simulink model "AUV_Multi_MPC"  (R2023a)
settings: Solver=ode23t  StartTime=0.0  StopTime=300  MaxStep=0.01  RelTol=1e-3  EnableMultiTasking=on
PreLoadFcn:
  | AUV_VehicleParameters;
  | Vehicle.Body.markeropacity = 0;
InitFcn:
  | %% ========================= SAMPLE TIME =========================
  | Ts = 0.1;
  | %% ========================= MPC: SURGE X =========================
  | nx = 1; nu = 1; ny = 1;
  | 
  | A = 0.9; B = 0.1; C = 1; D = 0;
  | plant = ss(A, B, C, D, Ts);
  | mpc1 = mpc(plant, Ts);
  | 
  | % Cấu hình như bình thường
  | mpc1.PredictionHorizon = 10;
  | mpc1.ControlHorizon = 2;
  | 
  | mpc1.Weights.OV = 7.5; % đủ mạnh để bám
  | mpc1.Weights.MV = 0.08; % cho dùng lực nhiều hơn
  | mpc1.Weights.MVRate = 0.25; % vừa mượt vừa linh hoạt
  | mpc1.MV.Min = -40;
  | mpc1.MV.Max = 40;
  | mpc1.OV.Min = 0;
  | mpc1.OV.Max = 2;
  | 
  | % Ràng buộc về thay đổi lực
  | mpc1.MV.RateMin = -12.5;
  | mpc1.MV.RateMax = 12.5;
  | %% ========================= MPC OUTER LOOP FOR DEPTH (Z) =========================
  | % ===== Baseline outer MPC for depth =====
  | u0 = 1.2;
  | 
  | A = 1;
  | B = -Ts*u0;
  | C = 1;
  | D = 0;
  | 
  | plant_z = ss(A,B,C,D,Ts);
  | 
  | mpc_z = mpc(plant_z,Ts);
  | mpc_z.PredictionHorizon = 10;
  | mpc_z.ControlHorizon    = 2;
  | 
  | mpc_z.Weights.OV     = 12;
  | mpc_z.Weights.MV     = 0.01;
  | mpc_z.Weights.MVRate = 0.1;
  | 
  | theta_ref_max = deg2rad(18);
  | mpc_z.MV.Min = -theta_ref_max;
  | mpc_z.MV.Max =  theta_ref_max;
  | 
  | mpc_z.MV.RateMin = -deg2rad(4);
  | mpc_z.MV.RateMax =  deg2rad(4);
  | 
  | 
  | %% ========================= MPC OUTER LOOP FOR HEADING =========================
  | A = 1;
  | B = Ts;
  | C = 1;
  | D = 0;
  | 
  | plant_psi = ss(A,B,C,D,Ts);
  | mpc_psi = mpc(plant_psi,Ts);
  | 
  | ... (+13 lines)
StopFcn:
  | try
  |     S = out;
  | 
  |     % ===============================
  |     % CHỌN HỆ QUY CHIẾU
  |     % ===============================
  |     USE_UP = true;   % true = ENU (Up), false = NED (Down)
  | 
  |     % ===============================
  |     % AUV position (NED gốc)
  |     % ===============================
  |     P  = squeeze(S.auv_position.signals.values);   % [Xn Ye Zd]
  |     tP = S.auv_position.time(:);
  | 
  |     Xn = P(:,1);   % North
  |     Ye = P(:,2);   % East
  |     Zd = P(:,3);   % Down (+)
  | 
  |     % ===============================
  |     % Reference vector
  |     % ===============================
  |     R = squeeze(S.auv_reference.signals.values);  % [V D psi]
  |     t = S.auv_reference.time(:);
  | 
  |     V   = R(:,1);      % speed
  |     D   = R(:,2);      % depth (Down +)
  |     psi = R(:,3);      % heading (rad)
  | 
  |     % ===============================
  |     % Reconstruct reference trajectory (NED)
  |     % ===============================
  |     Xr = Xn(1) + cumtrapz(t, V .* cos(psi));   % North
  |     Yr = Ye(1) + cumtrapz(t, V .* sin(psi));   % East
  |     Zr_down = Zd(1) + (D - D(1));              % Down (+)
  | 
  |     % ===============================
  |     % CHUYỂN HỆ (nếu cần)
  |     % ===============================
  |     if USE_UP
  |         Za  = -Zd;        % Up
  |         Zr  = -Zr_down;   % Up
  |         zlbl = 'Z (Up, m)';
  |     else
  |         Za  = Zd;         % Down
  |         Zr  = Zr_down;
  |         zlbl = 'Z (Down, m)';
  |     end
  | 
  |     % ===============================
  |     % Plot
  |     % ===============================
  |     f = figure(2); clf(f);
  |     set(f,'Name','AUV vs Reference','NumberTitle','off');
  | 
  |     ax = gca;
  |     ax.SortMethod = 'childorder';
  | 
  |     hRef   = plot3(Xr, Yr, Zr, '--', ...
  |                    'Color',[0.6 0.6 0.6], 'LineWidth',1.2);
  |     hold on
  | ... (+24 lines)
model workspace: external: MATLAB File AUV_DataFile_ORIG.m (data not in the file)
undefined symbols (not defined in the file): Environment, Multibody, Newton, Raphson, smiData, X, x, Y, y, Z
libraries: sm_lib x3123, nesl_utility x51, sharedutil x8, simulink x6, AUVCustomPrimitives_Lib x4, mpclib x3, fuzblock x2, instrumentseriallib x2, shared6dof x1, slpidlib x1, aerolibasang x1, aerolibadyn x1
(part 7 of 72)

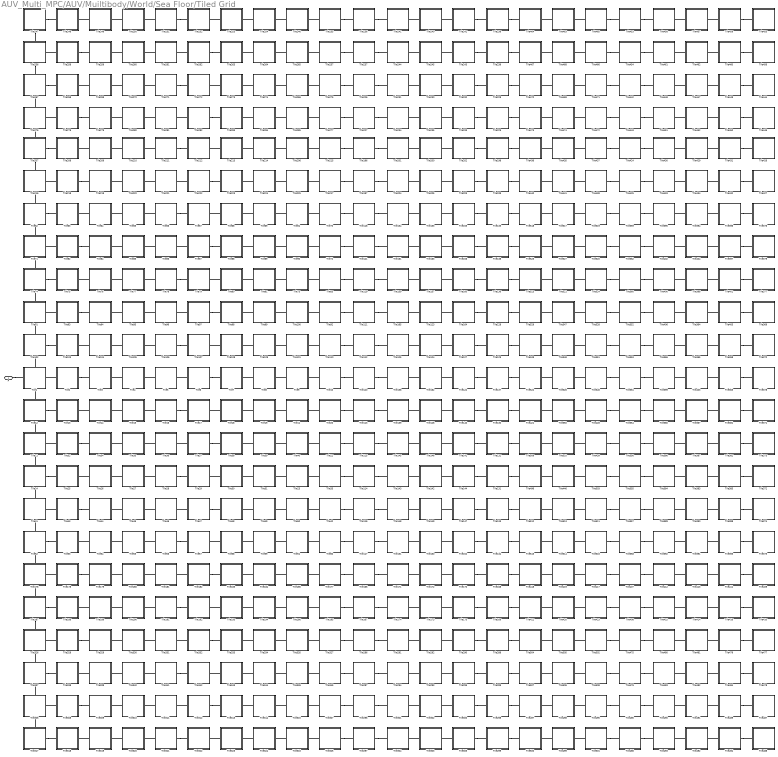
== system AUV_Multi_MPC/AUV/Muiltibody/World/Sea Floor/Tiled Grid ==
  Tile1 : Subsystem  mask(Square Tile){side=side, thickness=thick, color=color1, opacity=opacity}
      mask prompts: side "Side (m) :"; thickness "Thickness (m) :"; color "Color [RGB] :"; opacity "Opacity (0...1) :"
      mask help: This block creates a flat, single, square tile element. The square tile body is mass-less, so it will not have an effect on the dynamic simulation. This square tile element can be used as a graphic reference by itself, or as part of a composite graphic reference made of an array of interconnected tiles. The square tile is aligned with the XY plane, and the block provides frame connector ports to the middle points on each of the four sides of the body of the square - right (+X), left (-X), top (+Y) and bottom (-Y). All dimensions are in meters.
      settings: PortSchema="{\"entries\":[{\"content\":{\"sides\":[{\"content\":{\"connectorIds\":[\"LConn1\"]},\"type\":\"ConnectorPlacement.EquallySpacedRectSide\",\"uuid\":\"a971723f-ea37-4e9b-910b-501b94fb0ba2\"},{\"content\":{\"connectorIds\":[\"RConn1\"],\"side\":\"RIGHT\"},\"type\":\"ConnectorPlacement.EquallySpacedRectSide\",\"uuid\":\"e50175c1-005c-4b0b-bced-b882197eaab2\"},{\"content\":{\"connectorIds\":[\"LConn2\"],\"side\":\"TOP\"},\"type\":\"ConnectorPlacement.EquallySpacedRectSide\",\"uuid\":\"2a04a964-d53e-47ee-8c79-d53dd599bafe\"},{\"content\":{\"connectorIds\":[\"RConn2\"],\"side\":\"BOTTOM\"},\"type\":\"ConnectorPlacement.EquallySpacedRectSide\",\"uuid\":\"a0066dd6-a193-491c-afbe-bac00dfc3505\"}]},\"type\":\"ConnectorPlacement.EquallySpacedConnector\",\"uuid\":\"c80211c6-bb24-481b-97ca-2752015f3b18\"}],\"packageUris\":[\"http://schema.mathworks.com/mf0/Connector/19700101\"],\"version\":\"1.0\"}"
  Tile10 : Subsystem  mask(Square Tile){side=side, thickness=thick, color=color2, opacity=opacity}
      mask prompts: side "Side (m) :"; thickness "Thickness (m) :"; color "Color [RGB] :"; opacity "Opacity (0...1) :"
      mask help: This block creates a flat, single, square tile element. The square tile body is mass-less, so it will not have an effect on the dynamic simulation. This square tile element can be used as a graphic reference by itself, or as part of a composite graphic reference made of an array of interconnected tiles. The square tile is aligned with the XY plane, and the block provides frame connector ports to the middle points on each of the four sides of the body of the square - right (+X), left (-X), top (+Y) and bottom (-Y). All dimensions are in meters.
      settings: PortSchema="{\"entries\":[{\"content\":{\"sides\":[{\"content\":{\"connectorIds\":[\"LConn1\"]},\"type\":\"ConnectorPlacement.EquallySpacedRectSide\",\"uuid\":\"a971723f-ea37-4e9b-910b-501b94fb0ba2\"},{\"content\":{\"connectorIds\":[\"RConn1\"],\"side\":\"RIGHT\"},\"type\":\"ConnectorPlacement.EquallySpacedRectSide\",\"uuid\":\"e50175c1-005c-4b0b-bced-b882197eaab2\"},{\"content\":{\"connectorIds\":[\"LConn2\"],\"side\":\"TOP\"},\"type\":\"ConnectorPlacement.EquallySpacedRectSide\",\"uuid\":\"2a04a964-d53e-47ee-8c79-d53dd599bafe\"},{\"content\":{\"connectorIds\":[\"RConn2\"],\"side\":\"BOTTOM\"},\"type\":\"ConnectorPlacement.EquallySpacedRectSide\",\"uuid\":\"a0066dd6-a193-491c-afbe-bac00dfc3505\"}]},\"type\":\"ConnectorPlacement.EquallySpacedConnector\",\"uuid\":\"c80211c6-bb24-481b-97ca-2752015f3b18\"}],\"packageUris\":[\"http://schema.mathworks.com/mf0/Connector/19700101\"],\"version\":\"1.0\"}"
  Tile100 : Subsystem  mask(Square Tile){side=side, thickness=thick, color=color1, opacity=opacity}
      mask prompts: side "Side (m) :"; thickness "Thickness (m) :"; color "Color [RGB] :"; opacity "Opacity (0...1) :"
      mask help: This block creates a flat, single, square tile element. The square tile body is mass-less, so it will not have an effect on the dynamic simulation. This square tile element can be used as a graphic reference by itself, or as part of a composite graphic reference made of an array of interconnected tiles. The square tile is aligned with the XY plane, and the block provides frame connector ports to the middle points on each of the four sides of the body of the square - right (+X), left (-X), top (+Y) and bottom (-Y). All dimensions are in meters.
      settings: PortSchema="{\"entries\":[{\"content\":{\"sides\":[{\"content\":{\"connectorIds\":[\"LConn1\"]},\"type\":\"ConnectorPlacement.EquallySpacedRectSide\",\"uuid\":\"a971723f-ea37-4e9b-910b-501b94fb0ba2\"},{\"content\":{\"connectorIds\":[\"RConn1\"],\"side\":\"RIGHT\"},\"type\":\"ConnectorPlacement.EquallySpacedRectSide\",\"uuid\":\"e50175c1-005c-4b0b-bced-b882197eaab2\"},{\"content\":{\"connectorIds\":[\"LConn2\"],\"side\":\"TOP\"},\"type\":\"ConnectorPlacement.EquallySpacedRectSide\",\"uuid\":\"2a04a964-d53e-47ee-8c79-d53dd599bafe\"},{\"content\":{\"connectorIds\":[\"RConn2\"],\"side\":\"BOTTOM\"},\"type\":\"ConnectorPlacement.EquallySpacedRectSide\",\"uuid\":\"a0066dd6-a193-491c-afbe-bac00dfc3505\"}]},\"type\":\"ConnectorPlacement.EquallySpacedConnector\",\"uuid\":\"c80211c6-bb24-481b-97ca-2752015f3b18\"}],\"packageUris\":[\"http://schema.mathworks.com/mf0/Connector/19700101\"],\"version\":\"1.0\"}"
  Tile101 : Subsystem  mask(Square Tile){side=side, thickness=thick, color=color2, opacity=opacity}
      mask prompts: side "Side (m) :"; thickness "Thickness (m) :"; color "Color [RGB] :"; opacity "Opacity (0...1) :"
      mask help: This block creates a flat, single, square tile element. The square tile body is mass-less, so it will not have an effect on the dynamic simulation. This square tile element can be used as a graphic reference by itself, or as part of a composite graphic reference made of an array of interconnected tiles. The square tile is aligned with the XY plane, and the block provides frame connector ports to the middle points on each of the four sides of the body of the square - right (+X), left (-X), top (+Y) and bottom (-Y). All dimensions are in meters.
      settings: PortSchema="{\"entries\":[{\"content\":{\"sides\":[{\"content\":{\"connectorIds\":[\"LConn1\"]},\"type\":\"ConnectorPlacement.EquallySpacedRectSide\",\"uuid\":\"a971723f-ea37-4e9b-910b-501b94fb0ba2\"},{\"content\":{\"connectorIds\":[\"RConn1\"],\"side\":\"RIGHT\"},\"type\":\"ConnectorPlacement.EquallySpacedRectSide\",\"uuid\":\"e50175c1-005c-4b0b-bced-b882197eaab2\"},{\"content\":{\"connectorIds\":[\"LConn2\"],\"side\":\"TOP\"},\"type\":\"ConnectorPlacement.EquallySpacedRectSide\",\"uuid\":\"2a04a964-d53e-47ee-8c79-d53dd599bafe\"},{\"content\":{\"connectorIds\":[\"RConn2\"],\"side\":\"BOTTOM\"},\"type\":\"ConnectorPlacement.EquallySpacedRectSide\",\"uuid\":\"a0066dd6-a193-491c-afbe-bac00dfc3505\"}]},\"type\":\"ConnectorPlacement.EquallySpacedConnector\",\"uuid\":\"c80211c6-bb24-481b-97ca-2752015f3b18\"}],\"packageUris\":[\"http://schema.mathworks.com/mf0/Connector/19700101\"],\"version\":\"1.0\"}"
  Tile102 : Subsystem  mask(Square Tile){side=side, thickness=thick, color=color2, opacity=opacity}
      mask prompts: side "Side (m) :"; thickness "Thickness (m) :"; color "Color [RGB] :"; opacity "Opacity (0...1) :"
      mask help: This block creates a flat, single, square tile element. The square tile body is mass-less, so it will not have an effect on the dynamic simulation. This square tile element can be used as a graphic reference by itself, or as part of a composite graphic reference made of an array of interconnected tiles. The square tile is aligned with the XY plane, and the block provides frame connector ports to the middle points on each of the four sides of the body of the square - right (+X), left (-X), top (+Y) and bottom (-Y). All dimensions are in meters.
      settings: PortSchema="{\"entries\":[{\"content\":{\"sides\":[{\"content\":{\"connectorIds\":[\"LConn1\"]},\"type\":\"ConnectorPlacement.EquallySpacedRectSide\",\"uuid\":\"a971723f-ea37-4e9b-910b-501b94fb0ba2\"},{\"content\":{\"connectorIds\":[\"RConn1\"],\"side\":\"RIGHT\"},\"type\":\"ConnectorPlacement.EquallySpacedRectSide\",\"uuid\":\"e50175c1-005c-4b0b-bced-b882197eaab2\"},{\"content\":{\"connectorIds\":[\"LConn2\"],\"side\":\"TOP\"},\"type\":\"ConnectorPlacement.EquallySpacedRectSide\",\"uuid\":\"2a04a964-d53e-47ee-8c79-d53dd599bafe\"},{\"content\":{\"connectorIds\":[\"RConn2\"],\"side\":\"BOTTOM\"},\"type\":\"ConnectorPlacement.EquallySpacedRectSide\",\"uuid\":\"a0066dd6-a193-491c-afbe-bac00dfc3505\"}]},\"type\":\"ConnectorPlacement.EquallySpacedConnector\",\"uuid\":\"c80211c6-bb24-481b-97ca-2752015f3b18\"}],\"packageUris\":[\"http://schema.mathworks.com/mf0/Connector/19700101\"],\"version\":\"1.0\"}"
  Tile103 : Subsystem  mask(Square Tile){side=side, thickness=thick, color=color1, opacity=opacity}
      mask prompts: side "Side (m) :"; thickness "Thickness (m) :"; color "Color [RGB] :"; opacity "Opacity (0...1) :"
      mask help: This block creates a flat, single, square tile element. The square tile body is mass-less, so it will not have an effect on the dynamic simulation. This square tile element can be used as a graphic reference by itself, or as part of a composite graphic reference made of an array of interconnected tiles. The square tile is aligned with the XY plane, and the block provides frame connector ports to the middle points on each of the four sides of the body of the square - right (+X), left (-X), top (+Y) and bottom (-Y). All dimensions are in meters.
      settings: PortSchema="{\"entries\":[{\"content\":{\"sides\":[{\"content\":{\"connectorIds\":[\"LConn1\"]},\"type\":\"ConnectorPlacement.EquallySpacedRectSide\",\"uuid\":\"a971723f-ea37-4e9b-910b-501b94fb0ba2\"},{\"content\":{\"connectorIds\":[\"RConn1\"],\"side\":\"RIGHT\"},\"type\":\"ConnectorPlacement.EquallySpacedRectSide\",\"uuid\":\"e50175c1-005c-4b0b-bced-b882197eaab2\"},{\"content\":{\"connectorIds\":[\"LConn2\"],\"side\":\"TOP\"},\"type\":\"ConnectorPlacement.EquallySpacedRectSide\",\"uuid\":\"2a04a964-d53e-47ee-8c79-d53dd599bafe\"},{\"content\":{\"connectorIds\":[\"RConn2\"],\"side\":\"BOTTOM\"},\"type\":\"ConnectorPlacement.EquallySpacedRectSide\",\"uuid\":\"a0066dd6-a193-491c-afbe-bac00dfc3505\"}]},\"type\":\"ConnectorPlacement.EquallySpacedConnector\",\"uuid\":\"c80211c6-bb24-481b-97ca-2752015f3b18\"}],\"packageUris\":[\"http://schema.mathworks.com/mf0/Connector/19700101\"],\"version\":\"1.0\"}"
  Tile104 : Subsystem  mask(Square Tile){side=side, thickness=thick, color=color2, opacity=opacity}
      mask prompts: side "Side (m) :"; thickness "Thickness (m) :"; color "Color [RGB] :"; opacity "Opacity (0...1) :"
      mask help: This block creates a flat, single, square tile element. The square tile body is mass-less, so it will not have an effect on the dynamic simulation. This square tile element can be used as a graphic reference by itself, or as part of a composite graphic reference made of an array of interconnected tiles. The square tile is aligned with the XY plane, and the block provides frame connector ports to the middle points on each of the four sides of the body of the square - right (+X), left (-X), top (+Y) and bottom (-Y). All dimensions are in meters.
      settings: PortSchema="{\"entries\":[{\"content\":{\"sides\":[{\"content\":{\"connectorIds\":[\"LConn1\"]},\"type\":\"ConnectorPlacement.EquallySpacedRectSide\",\"uuid\":\"a971723f-ea37-4e9b-910b-501b94fb0ba2\"},{\"content\":{\"connectorIds\":[\"RConn1\"],\"side\":\"RIGHT\"},\"type\":\"ConnectorPlacement.EquallySpacedRectSide\",\"uuid\":\"e50175c1-005c-4b0b-bced-b882197eaab2\"},{\"content\":{\"connectorIds\":[\"LConn2\"],\"side\":\"TOP\"},\"type\":\"ConnectorPlacement.EquallySpacedRectSide\",\"uuid\":\"2a04a964-d53e-47ee-8c79-d53dd599bafe\"},{\"content\":{\"connectorIds\":[\"RConn2\"],\"side\":\"BOTTOM\"},\"type\":\"ConnectorPlacement.EquallySpacedRectSide\",\"uuid\":\"a0066dd6-a193-491c-afbe-bac00dfc3505\"}]},\"type\":\"ConnectorPlacement.EquallySpacedConnector\",\"uuid\":\"c80211c6-bb24-481b-97ca-2752015f3b18\"}],\"packageUris\":[\"http://schema.mathworks.com/mf0/Connector/19700101\"],\"version\":\"1.0\"}"
  Tile105 : Subsystem  mask(Square Tile){side=side, thickness=thick, color=color1, opacity=opacity}
      mask prompts: side "Side (m) :"; thickness "Thickness (m) :"; color "Color [RGB] :"; opacity "Opacity (0...1) :"
      mask help: This block creates a flat, single, square tile element. The square tile body is mass-less, so it will not have an effect on the dynamic simulation. This square tile element can be used as a graphic reference by itself, or as part of a composite graphic reference made of an array of interconnected tiles. The square tile is aligned with the XY plane, and the block provides frame connector ports to the middle points on each of the four sides of the body of the square - right (+X), left (-X), top (+Y) and bottom (-Y). All dimensions are in meters.
      settings: PortSchema="{\"entries\":[{\"content\":{\"sides\":[{\"content\":{\"connectorIds\":[\"LConn1\"]},\"type\":\"ConnectorPlacement.EquallySpacedRectSide\",\"uuid\":\"a971723f-ea37-4e9b-910b-501b94fb0ba2\"},{\"content\":{\"connectorIds\":[\"RConn1\"],\"side\":\"RIGHT\"},\"type\":\"ConnectorPlacement.EquallySpacedRectSide\",\"uuid\":\"e50175c1-005c-4b0b-bced-b882197eaab2\"},{\"content\":{\"connectorIds\":[\"LConn2\"],\"side\":\"TOP\"},\"type\":\"ConnectorPlacement.EquallySpacedRectSide\",\"uuid\":\"2a04a964-d53e-47ee-8c79-d53dd599bafe\"},{\"content\":{\"connectorIds\":[\"RConn2\"],\"side\":\"BOTTOM\"},\"type\":\"ConnectorPlacement.EquallySpacedRectSide\",\"uuid\":\"a0066dd6-a193-491c-afbe-bac00dfc3505\"}]},\"type\":\"ConnectorPlacement.EquallySpacedConnector\",\"uuid\":\"c80211c6-bb24-481b-97ca-2752015f3b18\"}],\"packageUris\":[\"http://schema.mathworks.com/mf0/Connector/19700101\"],\"version\":\"1.0\"}"
  Tile106 : Subsystem  mask(Square Tile){side=side, thickness=thick, color=color2, opacity=opacity}
      mask prompts: side "Side (m) :"; thickness "Thickness (m) :"; color "Color [RGB] :"; opacity "Opacity (0...1) :"
      mask help: This block creates a flat, single, square tile element. The square tile body is mass-less, so it will not have an effect on the dynamic simulation. This square tile element can be used as a graphic reference by itself, or as part of a composite graphic reference made of an array of interconnected tiles. The square tile is aligned with the XY plane, and the block provides frame connector ports to the middle points on each of the four sides of the body of the square - right (+X), left (-X), top (+Y) and bottom (-Y). All dimensions are in meters.
      settings: PortSchema="{\"entries\":[{\"content\":{\"sides\":[{\"content\":{\"connectorIds\":[\"LConn1\"]},\"type\":\"ConnectorPlacement.EquallySpacedRectSide\",\"uuid\":\"a971723f-ea37-4e9b-910b-501b94fb0ba2\"},{\"content\":{\"connectorIds\":[\"RConn1\"],\"side\":\"RIGHT\"},\"type\":\"ConnectorPlacement.EquallySpacedRectSide\",\"uuid\":\"e50175c1-005c-4b0b-bced-b882197eaab2\"},{\"content\":{\"connectorIds\":[\"LConn2\"],\"side\":\"TOP\"},\"type\":\"ConnectorPlacement.EquallySpacedRectSide\",\"uuid\":\"2a04a964-d53e-47ee-8c79-d53dd599bafe\"},{\"content\":{\"connectorIds\":[\"RConn2\"],\"side\":\"BOTTOM\"},\"type\":\"ConnectorPlacement.EquallySpacedRectSide\",\"uuid\":\"a0066dd6-a193-491c-afbe-bac00dfc3505\"}]},\"type\":\"ConnectorPlacement.EquallySpacedConnector\",\"uuid\":\"c80211c6-bb24-481b-97ca-2752015f3b18\"}],\"packageUris\":[\"http://schema.mathworks.com/mf0/Connector/19700101\"],\"version\":\"1.0\"}"
  Tile107 : Subsystem  mask(Square Tile){side=side, thickness=thick, color=color1, opacity=opacity}
      mask prompts: side "Side (m) :"; thickness "Thickness (m) :"; color "Color [RGB] :"; opacity "Opacity (0...1) :"
      mask help: This block creates a flat, single, square tile element. The square tile body is mass-less, so it will not have an effect on the dynamic simulation. This square tile element can be used as a graphic reference by itself, or as part of a composite graphic reference made of an array of interconnected tiles. The square tile is aligned with the XY plane, and the block provides frame connector ports to the middle points on each of the four sides of the body of the square - right (+X), left (-X), top (+Y) and bottom (-Y). All dimensions are in meters.
      settings: PortSchema="{\"entries\":[{\"content\":{\"sides\":[{\"content\":{\"connectorIds\":[\"LConn1\"]},\"type\":\"ConnectorPlacement.EquallySpacedRectSide\",\"uuid\":\"a971723f-ea37-4e9b-910b-501b94fb0ba2\"},{\"content\":{\"connectorIds\":[\"RConn1\"],\"side\":\"RIGHT\"},\"type\":\"ConnectorPlacement.EquallySpacedRectSide\",\"uuid\":\"e50175c1-005c-4b0b-bced-b882197eaab2\"},{\"content\":{\"connectorIds\":[\"LConn2\"],\"side\":\"TOP\"},\"type\":\"ConnectorPlacement.EquallySpacedRectSide\",\"uuid\":\"2a04a964-d53e-47ee-8c79-d53dd599bafe\"},{\"content\":{\"connectorIds\":[\"RConn2\"],\"side\":\"BOTTOM\"},\"type\":\"ConnectorPlacement.EquallySpacedRectSide\",\"uuid\":\"a0066dd6-a193-491c-afbe-bac00dfc3505\"}]},\"type\":\"ConnectorPlacement.EquallySpacedConnector\",\"uuid\":\"c80211c6-bb24-481b-97ca-2752015f3b18\"}],\"packageUris\":[\"http://schema.mathworks.com/mf0/Connector/19700101\"],\"version\":\"1.0\"}"
  Tile108 : Subsystem  mask(Square Tile){side=side, thickness=thick, color=color2, opacity=opacity}
      mask prompts: side "Side (m) :"; thickness "Thickness (m) :"; color "Color [RGB] :"; opacity "Opacity (0...1) :"
      mask help: This block creates a flat, single, square tile element. The square tile body is mass-less, so it will not have an effect on the dynamic simulation. This square tile element can be used as a graphic reference by itself, or as part of a composite graphic reference made of an array of interconnected tiles. The square tile is aligned with the XY plane, and the block provides frame connector ports to the middle points on each of the four sides of the body of the square - right (+X), left (-X), top (+Y) and bottom (-Y). All dimensions are in meters.
      settings: PortSchema="{\"entries\":[{\"content\":{\"sides\":[{\"content\":{\"connectorIds\":[\"LConn1\"]},\"type\":\"ConnectorPlacement.EquallySpacedRectSide\",\"uuid\":\"a971723f-ea37-4e9b-910b-501b94fb0ba2\"},{\"content\":{\"connectorIds\":[\"RConn1\"],\"side\":\"RIGHT\"},\"type\":\"ConnectorPlacement.EquallySpacedRectSide\",\"uuid\":\"e50175c1-005c-4b0b-bced-b882197eaab2\"},{\"content\":{\"connectorIds\":[\"LConn2\"],\"side\":\"TOP\"},\"type\":\"ConnectorPlacement.EquallySpacedRectSide\",\"uuid\":\"2a04a964-d53e-47ee-8c79-d53dd599bafe\"},{\"content\":{\"connectorIds\":[\"RConn2\"],\"side\":\"BOTTOM\"},\"type\":\"ConnectorPlacement.EquallySpacedRectSide\",\"uuid\":\"a0066dd6-a193-491c-afbe-bac00dfc3505\"}]},\"type\":\"ConnectorPlacement.EquallySpacedConnector\",\"uuid\":\"c80211c6-bb24-481b-97ca-2752015f3b18\"}],\"packageUris\":[\"http://schema.mathworks.com/mf0/Connector/19700101\"],\"version\":\"1.0\"}"
  Tile109 : Subsystem  mask(Square Tile){side=side, thickness=thick, color=color1, opacity=opacity}
      mask prompts: side "Side (m) :"; thickness "Thickness (m) :"; color "Color [RGB] :"; opacity "Opacity (0...1) :"
      mask help: This block creates a flat, single, square tile element. The square tile body is mass-less, so it will not have an effect on the dynamic simulation. This square tile element can be used as a graphic reference by itself, or as part of a composite graphic reference made of an array of interconnected tiles. The square tile is aligned with the XY plane, and the block provides frame connector ports to the middle points on each of the four sides of the body of the square - right (+X), left (-X), top (+Y) and bottom (-Y). All dimensions are in meters.
      settings: PortSchema="{\"entries\":[{\"content\":{\"sides\":[{\"content\":{\"connectorIds\":[\"LConn1\"]},\"type\":\"ConnectorPlacement.EquallySpacedRectSide\",\"uuid\":\"a971723f-ea37-4e9b-910b-501b94fb0ba2\"},{\"content\":{\"connectorIds\":[\"RConn1\"],\"side\":\"RIGHT\"},\"type\":\"ConnectorPlacement.EquallySpacedRectSide\",\"uuid\":\"e50175c1-005c-4b0b-bced-b882197eaab2\"},{\"content\":{\"connectorIds\":[\"LConn2\"],\"side\":\"TOP\"},\"type\":\"ConnectorPlacement.EquallySpacedRectSide\",\"uuid\":\"2a04a964-d53e-47ee-8c79-d53dd599bafe\"},{\"content\":{\"connectorIds\":[\"RConn2\"],\"side\":\"BOTTOM\"},\"type\":\"ConnectorPlacement.EquallySpacedRectSide\",\"uuid\":\"a0066dd6-a193-491c-afbe-bac00dfc3505\"}]},\"type\":\"ConnectorPlacement.EquallySpacedConnector\",\"uuid\":\"c80211c6-bb24-481b-97ca-2752015f3b18\"}],\"packageUris\":[\"http://schema.mathworks.com/mf0/Connector/19700101\"],\"version\":\"1.0\"}"
  Tile11 : Subsystem  mask(Square Tile){side=side, thickness=thick, color=color2, opacity=opacity}
      mask prompts: side "Side (m) :"; thickness "Thickness (m) :"; color "Color [RGB] :"; opacity "Opacity (0...1) :"
      mask help: This block creates a flat, single, square tile element. The square tile body is mass-less, so it will not have an effect on the dynamic simulation. This square tile element can be used as a graphic reference by itself, or as part of a composite graphic reference made of an array of interconnected tiles. The square tile is aligned with the XY plane, and the block provides frame connector ports to the middle points on each of the four sides of the body of the square - right (+X), left (-X), top (+Y) and bottom (-Y). All dimensions are in meters.
      settings: PortSchema="{\"entries\":[{\"content\":{\"sides\":[{\"content\":{\"connectorIds\":[\"LConn1\"]},\"type\":\"ConnectorPlacement.EquallySpacedRectSide\",\"uuid\":\"a971723f-ea37-4e9b-910b-501b94fb0ba2\"},{\"content\":{\"connectorIds\":[\"RConn1\"],\"side\":\"RIGHT\"},\"type\":\"ConnectorPlacement.EquallySpacedRectSide\",\"uuid\":\"e50175c1-005c-4b0b-bced-b882197eaab2\"},{\"content\":{\"connectorIds\":[\"LConn2\"],\"side\":\"TOP\"},\"type\":\"ConnectorPlacement.EquallySpacedRectSide\",\"uuid\":\"2a04a964-d53e-47ee-8c79-d53dd599bafe\"},{\"content\":{\"connectorIds\":[\"RConn2\"],\"side\":\"BOTTOM\"},\"type\":\"ConnectorPlacement.EquallySpacedRectSide\",\"uuid\":\"a0066dd6-a193-491c-afbe-bac00dfc3505\"}]},\"type\":\"ConnectorPlacement.EquallySpacedConnector\",\"uuid\":\"c80211c6-bb24-481b-97ca-2752015f3b18\"}],\"packageUris\":[\"http://schema.mathworks.com/mf0/Connector/19700101\"],\"version\":\"1.0\"}"
  Tile110 : Subsystem  mask(Square Tile){side=side, thickness=thick, color=color1, opacity=opacity}
      mask prompts: side "Side (m) :"; thickness "Thickness (m) :"; color "Color [RGB] :"; opacity "Opacity (0...1) :"
      mask help: This block creates a flat, single, square tile element. The square tile body is mass-less, so it will not have an effect on the dynamic simulation. This square tile element can be used as a graphic reference by itself, or as part of a composite graphic reference made of an array of interconnected tiles. The square tile is aligned with the XY plane, and the block provides frame connector ports to the middle points on each of the four sides of the body of the square - right (+X), left (-X), top (+Y) and bottom (-Y). All dimensions are in meters.
      settings: PortSchema="{\"entries\":[{\"content\":{\"sides\":[{\"content\":{\"connectorIds\":[\"LConn1\"]},\"type\":\"ConnectorPlacement.EquallySpacedRectSide\",\"uuid\":\"a971723f-ea37-4e9b-910b-501b94fb0ba2\"},{\"content\":{\"connectorIds\":[\"RConn1\"],\"side\":\"RIGHT\"},\"type\":\"ConnectorPlacement.EquallySpacedRectSide\",\"uuid\":\"e50175c1-005c-4b0b-bced-b882197eaab2\"},{\"content\":{\"connectorIds\":[\"LConn2\"],\"side\":\"TOP\"},\"type\":\"ConnectorPlacement.EquallySpacedRectSide\",\"uuid\":\"2a04a964-d53e-47ee-8c79-d53dd599bafe\"},{\"content\":{\"connectorIds\":[\"RConn2\"],\"side\":\"BOTTOM\"},\"type\":\"ConnectorPlacement.EquallySpacedRectSide\",\"uuid\":\"a0066dd6-a193-491c-afbe-bac00dfc3505\"}]},\"type\":\"ConnectorPlacement.EquallySpacedConnector\",\"uuid\":\"c80211c6-bb24-481b-97ca-2752015f3b18\"}],\"packageUris\":[\"http://schema.mathworks.com/mf0/Connector/19700101\"],\"version\":\"1.0\"}"
  Tile111 : Subsystem  mask(Square Tile){side=side, thickness=thick, color=color1, opacity=opacity}
      mask prompts: side "Side (m) :"; thickness "Thickness (m) :"; color "Color [RGB] :"; opacity "Opacity (0...1) :"
      mask help: This block creates a flat, single, square tile element. The square tile body is mass-less, so it will not have an effect on the dynamic simulation. This square tile element can be used as a graphic reference by itself, or as part of a composite graphic reference made of an array of interconnected tiles. The square tile is aligned with the XY plane, and the block provides frame connector ports to the middle points on each of the four sides of the body of the square - right (+X), left (-X), top (+Y) and bottom (-Y). All dimensions are in meters.
      settings: PortSchema="{\"entries\":[{\"content\":{\"sides\":[{\"content\":{\"connectorIds\":[\"LConn1\"]},\"type\":\"ConnectorPlacement.EquallySpacedRectSide\",\"uuid\":\"a971723f-ea37-4e9b-910b-501b94fb0ba2\"},{\"content\":{\"connectorIds\":[\"RConn1\"],\"side\":\"RIGHT\"},\"type\":\"ConnectorPlacement.EquallySpacedRectSide\",\"uuid\":\"e50175c1-005c-4b0b-bced-b882197eaab2\"},{\"content\":{\"connectorIds\":[\"LConn2\"],\"side\":\"TOP\"},\"type\":\"ConnectorPlacement.EquallySpacedRectSide\",\"uuid\":\"2a04a964-d53e-47ee-8c79-d53dd599bafe\"},{\"content\":{\"connectorIds\":[\"RConn2\"],\"side\":\"BOTTOM\"},\"type\":\"ConnectorPlacement.EquallySpacedRectSide\",\"uuid\":\"a0066dd6-a193-491c-afbe-bac00dfc3505\"}]},\"type\":\"ConnectorPlacement.EquallySpacedConnector\",\"uuid\":\"c80211c6-bb24-481b-97ca-2752015f3b18\"}],\"packageUris\":[\"http://schema.mathworks.com/mf0/Connector/19700101\"],\"version\":\"1.0\"}"
  Tile112 : Subsystem  mask(Square Tile){side=side, thickness=thick, color=color2, opacity=opacity}
      mask prompts: side "Side (m) :"; thickness "Thickness (m) :"; color "Color [RGB] :"; opacity "Opacity (0...1) :"
      mask help: This block creates a flat, single, square tile element. The square tile body is mass-less, so it will not have an effect on the dynamic simulation. This square tile element can be used as a graphic reference by itself, or as part of a composite graphic reference made of an array of interconnected tiles. The square tile is aligned with the XY plane, and the block provides frame connector ports to the middle points on each of the four sides of the body of the square - right (+X), left (-X), top (+Y) and bottom (-Y). All dimensions are in meters.
      settings: PortSchema="{\"entries\":[{\"content\":{\"sides\":[{\"content\":{\"connectorIds\":[\"LConn1\"]},\"type\":\"ConnectorPlacement.EquallySpacedRectSide\",\"uuid\":\"a971723f-ea37-4e9b-910b-501b94fb0ba2\"},{\"content\":{\"connectorIds\":[\"RConn1\"],\"side\":\"RIGHT\"},\"type\":\"ConnectorPlacement.EquallySpacedRectSide\",\"uuid\":\"e50175c1-005c-4b0b-bced-b882197eaab2\"},{\"content\":{\"connectorIds\":[\"LConn2\"],\"side\":\"TOP\"},\"type\":\"ConnectorPlacement.EquallySpacedRectSide\",\"uuid\":\"2a04a964-d53e-47ee-8c79-d53dd599bafe\"},{\"content\":{\"connectorIds\":[\"RConn2\"],\"side\":\"BOTTOM\"},\"type\":\"ConnectorPlacement.EquallySpacedRectSide\",\"uuid\":\"a0066dd6-a193-491c-afbe-bac00dfc3505\"}]},\"type\":\"ConnectorPlacement.EquallySpacedConnector\",\"uuid\":\"c80211c6-bb24-481b-97ca-2752015f3b18\"}],\"packageUris\":[\"http://schema.mathworks.com/mf0/Connector/19700101\"],\"version\":\"1.0\"}"
  Tile113 : Subsystem  mask(Square Tile){side=side, thickness=thick, color=color2, opacity=opacity}
      mask prompts: side "Side (m) :"; thickness "Thickness (m) :"; color "Color [RGB] :"; opacity "Opacity (0...1) :"
      mask help: This block creates a flat, single, square tile element. The square tile body is mass-less, so it will not have an effect on the dynamic simulation. This square tile element can be used as a graphic reference by itself, or as part of a composite graphic reference made of an array of interconnected tiles. The square tile is aligned with the XY plane, and the block provides frame connector ports to the middle points on each of the four sides of the body of the square - right (+X), left (-X), top (+Y) and bottom (-Y). All dimensions are in meters.
      settings: PortSchema="{\"entries\":[{\"content\":{\"sides\":[{\"content\":{\"connectorIds\":[\"LConn1\"]},\"type\":\"ConnectorPlacement.EquallySpacedRectSide\",\"uuid\":\"a971723f-ea37-4e9b-910b-501b94fb0ba2\"},{\"content\":{\"connectorIds\":[\"RConn1\"],\"side\":\"RIGHT\"},\"type\":\"ConnectorPlacement.EquallySpacedRectSide\",\"uuid\":\"e50175c1-005c-4b0b-bced-b882197eaab2\"},{\"content\":{\"connectorIds\":[\"LConn2\"],\"side\":\"TOP\"},\"type\":\"ConnectorPlacement.EquallySpacedRectSide\",\"uuid\":\"2a04a964-d53e-47ee-8c79-d53dd599bafe\"},{\"content\":{\"connectorIds\":[\"RConn2\"],\"side\":\"BOTTOM\"},\"type\":\"ConnectorPlacement.EquallySpacedRectSide\",\"uuid\":\"a0066dd6-a193-491c-afbe-bac00dfc3505\"}]},\"type\":\"ConnectorPlacement.EquallySpacedConnector\",\"uuid\":\"c80211c6-bb24-481b-97ca-2752015f3b18\"}],\"packageUris\":[\"http://schema.mathworks.com/mf0/Connector/19700101\"],\"version\":\"1.0\"}"
  Tile114 : Subsystem  mask(Square Tile){side=side, thickness=thick, color=color2, opacity=opacity}
      mask prompts: side "Side (m) :"; thickness "Thickness (m) :"; color "Color [RGB] :"; opacity "Opacity (0...1) :"
      mask help: This block creates a flat, single, square tile element. The square tile body is mass-less, so it will not have an effect on the dynamic simulation. This square tile element can be used as a graphic reference by itself, or as part of a composite graphic reference made of an array of interconnected tiles. The square tile is aligned with the XY plane, and the block provides frame connector ports to the middle points on each of the four sides of the body of the square - right (+X), left (-X), top (+Y) and bottom (-Y). All dimensions are in meters.
      settings: PortSchema="{\"entries\":[{\"content\":{\"sides\":[{\"content\":{\"connectorIds\":[\"LConn1\"]},\"type\":\"ConnectorPlacement.EquallySpacedRectSide\",\"uuid\":\"a971723f-ea37-4e9b-910b-501b94fb0ba2\"},{\"content\":{\"connectorIds\":[\"RConn1\"],\"side\":\"RIGHT\"},\"type\":\"ConnectorPlacement.EquallySpacedRectSide\",\"uuid\":\"e50175c1-005c-4b0b-bced-b882197eaab2\"},{\"content\":{\"connectorIds\":[\"LConn2\"],\"side\":\"TOP\"},\"type\":\"ConnectorPlacement.EquallySpacedRectSide\",\"uuid\":\"2a04a964-d53e-47ee-8c79-d53dd599bafe\"},{\"content\":{\"connectorIds\":[\"RConn2\"],\"side\":\"BOTTOM\"},\"type\":\"ConnectorPlacement.EquallySpacedRectSide\",\"uuid\":\"a0066dd6-a193-491c-afbe-bac00dfc3505\"}]},\"type\":\"ConnectorPlacement.EquallySpacedConnector\",\"uuid\":\"c80211c6-bb24-481b-97ca-2752015f3b18\"}],\"packageUris\":[\"http://schema.mathworks.com/mf0/Connector/19700101\"],\"version\":\"1.0\"}"
  Tile115 : Subsystem  mask(Square Tile){side=side, thickness=thick, color=color1, opacity=opacity}
      mask prompts: side "Side (m) :"; thickness "Thickness (m) :"; color "Color [RGB] :"; opacity "Opacity (0...1) :"
      mask help: This block creates a flat, single, square tile element. The square tile body is mass-less, so it will not have an effect on the dynamic simulation. This square tile element can be used as a graphic reference by itself, or as part of a composite graphic reference made of an array of interconnected tiles. The square tile is aligned with the XY plane, and the block provides frame connector ports to the middle points on each of the four sides of the body of the square - right (+X), left (-X), top (+Y) and bottom (-Y). All dimensions are in meters.
      settings: PortSchema="{\"entries\":[{\"content\":{\"sides\":[{\"content\":{\"connectorIds\":[\"LConn1\"]},\"type\":\"ConnectorPlacement.EquallySpacedRectSide\",\"uuid\":\"a971723f-ea37-4e9b-910b-501b94fb0ba2\"},{\"content\":{\"connectorIds\":[\"RConn1\"],\"side\":\"RIGHT\"},\"type\":\"ConnectorPlacement.EquallySpacedRectSide\",\"uuid\":\"e50175c1-005c-4b0b-bced-b882197eaab2\"},{\"content\":{\"connectorIds\":[\"LConn2\"],\"side\":\"TOP\"},\"type\":\"ConnectorPlacement.EquallySpacedRectSide\",\"uuid\":\"2a04a964-d53e-47ee-8c79-d53dd599bafe\"},{\"content\":{\"connectorIds\":[\"RConn2\"],\"side\":\"BOTTOM\"},\"type\":\"ConnectorPlacement.EquallySpacedRectSide\",\"uuid\":\"a0066dd6-a193-491c-afbe-bac00dfc3505\"}]},\"type\":\"ConnectorPlacement.EquallySpacedConnector\",\"uuid\":\"c80211c6-bb24-481b-97ca-2752015f3b18\"}],\"packageUris\":[\"http://schema.mathworks.com/mf0/Connector/19700101\"],\"version\":\"1.0\"}"
  Tile116 : Subsystem  mask(Square Tile){side=side, thickness=thick, color=color1, opacity=opacity}
      mask prompts: side "Side (m) :"; thickness "Thickness (m) :"; color "Color [RGB] :"; opacity "Opacity (0...1) :"
      mask help: This block creates a flat, single, square tile element. The square tile body is mass-less, so it will not have an effect on the dynamic simulation. This square tile element can be used as a graphic reference by itself, or as part of a composite graphic reference made of an array of interconnected tiles. The square tile is aligned with the XY plane, and the block provides frame connector ports to the middle points on each of the four sides of the body of the square - right (+X), left (-X), top (+Y) and bottom (-Y). All dimensions are in meters.
      settings: PortSchema="{\"entries\":[{\"content\":{\"sides\":[{\"content\":{\"connectorIds\":[\"LConn1\"]},\"type\":\"ConnectorPlacement.EquallySpacedRectSide\",\"uuid\":\"a971723f-ea37-4e9b-910b-501b94fb0ba2\"},{\"content\":{\"connectorIds\":[\"RConn1\"],\"side\":\"RIGHT\"},\"type\":\"ConnectorPlacement.EquallySpacedRectSide\",\"uuid\":\"e50175c1-005c-4b0b-bced-b882197eaab2\"},{\"content\":{\"connectorIds\":[\"LConn2\"],\"side\":\"TOP\"},\"type\":\"ConnectorPlacement.EquallySpacedRectSide\",\"uuid\":\"2a04a964-d53e-47ee-8c79-d53dd599bafe\"},{\"content\":{\"connectorIds\":[\"RConn2\"],\"side\":\"BOTTOM\"},\"type\":\"ConnectorPlacement.EquallySpacedRectSide\",\"uuid\":\"a0066dd6-a193-491c-afbe-bac00dfc3505\"}]},\"type\":\"ConnectorPlacement.EquallySpacedConnector\",\"uuid\":\"c80211c6-bb24-481b-97ca-2752015f3b18\"}],\"packageUris\":[\"http://schema.mathworks.com/mf0/Connector/19700101\"],\"version\":\"1.0\"}"
  Tile117 : Subsystem  mask(Square Tile){side=side, thickness=thick, color=color2, opacity=opacity}
      mask prompts: side "Side (m) :"; thickness "Thickness (m) :"; color "Color [RGB] :"; opacity "Opacity (0...1) :"
      mask help: This block creates a flat, single, square tile element. The square tile body is mass-less, so it will not have an effect on the dynamic simulation. This square tile element can be used as a graphic reference by itself, or as part of a composite graphic reference made of an array of interconnected tiles. The square tile is aligned with the XY plane, and the block provides frame connector ports to the middle points on each of the four sides of the body of the square - right (+X), left (-X), top (+Y) and bottom (-Y). All dimensions are in meters.
      settings: PortSchema="{\"entries\":[{\"content\":{\"sides\":[{\"content\":{\"connectorIds\":[\"LConn1\"]},\"type\":\"ConnectorPlacement.EquallySpacedRectSide\",\"uuid\":\"a971723f-ea37-4e9b-910b-501b94fb0ba2\"},{\"content\":{\"connectorIds\":[\"RConn1\"],\"side\":\"RIGHT\"},\"type\":\"ConnectorPlacement.EquallySpacedRectSide\",\"uuid\":\"e50175c1-005c-4b0b-bced-b882197eaab2\"},{\"content\":{\"connectorIds\":[\"LConn2\"],\"side\":\"TOP\"},\"type\":\"ConnectorPlacement.EquallySpacedRectSide\",\"uuid\":\"2a04a964-d53e-47ee-8c79-d53dd599bafe\"},{\"content\":{\"connectorIds\":[\"RConn2\"],\"side\":\"BOTTOM\"},\"type\":\"ConnectorPlacement.EquallySpacedRectSide\",\"uuid\":\"a0066dd6-a193-491c-afbe-bac00dfc3505\"}]},\"type\":\"ConnectorPlacement.EquallySpacedConnector\",\"uuid\":\"c80211c6-bb24-481b-97ca-2752015f3b18\"}],\"packageUris\":[\"http://schema.mathworks.com/mf0/Connector/19700101\"],\"version\":\"1.0\"}"
  Tile118 : Subsystem  mask(Square Tile){side=side, thickness=thick, color=color2, opacity=opacity}
      mask prompts: side "Side (m) :"; thickness "Thickness (m) :"; color "Color [RGB] :"; opacity "Opacity (0...1) :"
      mask help: This block creates a flat, single, square tile element. The square tile body is mass-less, so it will not have an effect on the dynamic simulation. This square tile element can be used as a graphic reference by itself, or as part of a composite graphic reference made of an array of interconnected tiles. The square tile is aligned with the XY plane, and the block provides frame connector ports to the middle points on each of the four sides of the body of the square - right (+X), left (-X), top (+Y) and bottom (-Y). All dimensions are in meters.
      settings: PortSchema="{\"entries\":[{\"content\":{\"sides\":[{\"content\":{\"connectorIds\":[\"LConn1\"]},\"type\":\"ConnectorPlacement.EquallySpacedRectSide\",\"uuid\":\"a971723f-ea37-4e9b-910b-501b94fb0ba2\"},{\"content\":{\"connectorIds\":[\"RConn1\"],\"side\":\"RIGHT\"},\"type\":\"ConnectorPlacement.EquallySpacedRectSide\",\"uuid\":\"e50175c1-005c-4b0b-bced-b882197eaab2\"},{\"content\":{\"connectorIds\":[\"LConn2\"],\"side\":\"TOP\"},\"type\":\"ConnectorPlacement.EquallySpacedRectSide\",\"uuid\":\"2a04a964-d53e-47ee-8c79-d53dd599bafe\"},{\"content\":{\"connectorIds\":[\"RConn2\"],\"side\":\"BOTTOM\"},\"type\":\"ConnectorPlacement.EquallySpacedRectSide\",\"uuid\":\"a0066dd6-a193-491c-afbe-bac00dfc3505\"}]},\"type\":\"ConnectorPlacement.EquallySpacedConnector\",\"uuid\":\"c80211c6-bb24-481b-97ca-2752015f3b18\"}],\"packageUris\":[\"http://schema.mathworks.com/mf0/Connector/19700101\"],\"version\":\"1.0\"}"
  Tile119 : Subsystem  mask(Square Tile){side=side, thickness=thick, color=color2, opacity=opacity}
      mask prompts: side "Side (m) :"; thickness "Thickness (m) :"; color "Color [RGB] :"; opacity "Opacity (0...1) :"
      mask help: This block creates a flat, single, square tile element. The square tile body is mass-less, so it will not have an effect on the dynamic simulation. This square tile element can be used as a graphic reference by itself, or as part of a composite graphic reference made of an array of interconnected tiles. The square tile is aligned with the XY plane, and the block provides frame connector ports to the middle points on each of the four sides of the body of the square - right (+X), left (-X), top (+Y) and bottom (-Y). All dimensions are in meters.
      settings: PortSchema="{\"entries\":[{\"content\":{\"sides\":[{\"content\":{\"connectorIds\":[\"LConn1\"]},\"type\":\"ConnectorPlacement.EquallySpacedRectSide\",\"uuid\":\"a971723f-ea37-4e9b-910b-501b94fb0ba2\"},{\"content\":{\"connectorIds\":[\"RConn1\"],\"side\":\"RIGHT\"},\"type\":\"ConnectorPlacement.EquallySpacedRectSide\",\"uuid\":\"e50175c1-005c-4b0b-bced-b882197eaab2\"},{\"content\":{\"connectorIds\":[\"LConn2\"],\"side\":\"TOP\"},\"type\":\"ConnectorPlacement.EquallySpacedRectSide\",\"uuid\":\"2a04a964-d53e-47ee-8c79-d53dd599bafe\"},{\"content\":{\"connectorIds\":[\"RConn2\"],\"side\":\"BOTTOM\"},\"type\":\"ConnectorPlacement.EquallySpacedRectSide\",\"uuid\":\"a0066dd6-a193-491c-afbe-bac00dfc3505\"}]},\"type\":\"ConnectorPlacement.EquallySpacedConnector\",\"uuid\":\"c80211c6-bb24-481b-97ca-2752015f3b18\"}],\"packageUris\":[\"http://schema.mathworks.com/mf0/Connector/19700101\"],\"version\":\"1.0\"}"
  Tile12 : Subsystem  mask(Square Tile){side=side, thickness=thick, color=color2, opacity=opacity}
      mask prompts: side "Side (m) :"; thickness "Thickness (m) :"; color "Color [RGB] :"; opacity "Opacity (0...1) :"
      mask help: This block creates a flat, single, square tile element. The square tile body is mass-less, so it will not have an effect on the dynamic simulation. This square tile element can be used as a graphic reference by itself, or as part of a composite graphic reference made of an array of interconnected tiles. The square tile is aligned with the XY plane, and the block provides frame connector ports to the middle points on each of the four sides of the body of the square - right (+X), left (-X), top (+Y) and bottom (-Y). All dimensions are in meters.
      settings: PortSchema="{\"entries\":[{\"content\":{\"sides\":[{\"content\":{\"connectorIds\":[\"LConn1\"]},\"type\":\"ConnectorPlacement.EquallySpacedRectSide\",\"uuid\":\"a971723f-ea37-4e9b-910b-501b94fb0ba2\"},{\"content\":{\"connectorIds\":[\"RConn1\"],\"side\":\"RIGHT\"},\"type\":\"ConnectorPlacement.EquallySpacedRectSide\",\"uuid\":\"e50175c1-005c-4b0b-bced-b882197eaab2\"},{\"content\":{\"connectorIds\":[\"LConn2\"],\"side\":\"TOP\"},\"type\":\"ConnectorPlacement.EquallySpacedRectSide\",\"uuid\":\"2a04a964-d53e-47ee-8c79-d53dd599bafe\"},{\"content\":{\"connectorIds\":[\"RConn2\"],\"side\":\"BOTTOM\"},\"type\":\"ConnectorPlacement.EquallySpacedRectSide\",\"uuid\":\"a0066dd6-a193-491c-afbe-bac00dfc3505\"}]},\"type\":\"ConnectorPlacement.EquallySpacedConnector\",\"uuid\":\"c80211c6-bb24-481b-97ca-2752015f3b18\"}],\"packageUris\":[\"http://schema.mathworks.com/mf0/Connector/19700101\"],\"version\":\"1.0\"}"
  Tile120 : Subsystem  mask(Square Tile){side=side, thickness=thick, color=color1, opacity=opacity}
      mask prompts: side "Side (m) :"; thickness "Thickness (m) :"; color "Color [RGB] :"; opacity "Opacity (0...1) :"
      mask help: This block creates a flat, single, square tile element. The square tile body is mass-less, so it will not have an effect on the dynamic simulation. This square tile element can be used as a graphic reference by itself, or as part of a composite graphic reference made of an array of interconnected tiles. The square tile is aligned with the XY plane, and the block provides frame connector ports to the middle points on each of the four sides of the body of the square - right (+X), left (-X), top (+Y) and bottom (-Y). All dimensions are in meters.
      settings: PortSchema="{\"entries\":[{\"content\":{\"sides\":[{\"content\":{\"connectorIds\":[\"LConn1\"]},\"type\":\"ConnectorPlacement.EquallySpacedRectSide\",\"uuid\":\"a971723f-ea37-4e9b-910b-501b94fb0ba2\"},{\"content\":{\"connectorIds\":[\"RConn1\"],\"side\":\"RIGHT\"},\"type\":\"ConnectorPlacement.EquallySpacedRectSide\",\"uuid\":\"e50175c1-005c-4b0b-bced-b882197eaab2\"},{\"content\":{\"connectorIds\":[\"LConn2\"],\"side\":\"TOP\"},\"type\":\"ConnectorPlacement.EquallySpacedRectSide\",\"uuid\":\"2a04a964-d53e-47ee-8c79-d53dd599bafe\"},{\"content\":{\"connectorIds\":[\"RConn2\"],\"side\":\"BOTTOM\"},\"type\":\"ConnectorPlacement.EquallySpacedRectSide\",\"uuid\":\"a0066dd6-a193-491c-afbe-bac00dfc3505\"}]},\"type\":\"ConnectorPlacement.EquallySpacedConnector\",\"uuid\":\"c80211c6-bb24-481b-97ca-2752015f3b18\"}],\"packageUris\":[\"http://schema.mathworks.com/mf0/Connector/19700101\"],\"version\":\"1.0\"}"
  Tile121 : Subsystem  mask(Square Tile){side=side, thickness=thick, color=color1, opacity=opacity}
      mask prompts: side "Side (m) :"; thickness "Thickness (m) :"; color "Color [RGB] :"; opacity "Opacity (0...1) :"
      mask help: This block creates a flat, single, square tile element. The square tile body is mass-less, so it will not have an effect on the dynamic simulation. This square tile element can be used as a graphic reference by itself, or as part of a composite graphic reference made of an array of interconnected tiles. The square tile is aligned with the XY plane, and the block provides frame connector ports to the middle points on each of the four sides of the body of the square - right (+X), left (-X), top (+Y) and bottom (-Y). All dimensions are in meters.
      settings: PortSchema="{\"entries\":[{\"content\":{\"sides\":[{\"content\":{\"connectorIds\":[\"LConn1\"]},\"type\":\"ConnectorPlacement.EquallySpacedRectSide\",\"uuid\":\"a971723f-ea37-4e9b-910b-501b94fb0ba2\"},{\"content\":{\"connectorIds\":[\"RConn1\"],\"side\":\"RIGHT\"},\"type\":\"ConnectorPlacement.EquallySpacedRectSide\",\"uuid\":\"e50175c1-005c-4b0b-bced-b882197eaab2\"},{\"content\":{\"connectorIds\":[\"LConn2\"],\"side\":\"TOP\"},\"type\":\"ConnectorPlacement.EquallySpacedRectSide\",\"uuid\":\"2a04a964-d53e-47ee-8c79-d53dd599bafe\"},{\"content\":{\"connectorIds\":[\"RConn2\"],\"side\":\"BOTTOM\"},\"type\":\"ConnectorPlacement.EquallySpacedRectSide\",\"uuid\":\"a0066dd6-a193-491c-afbe-bac00dfc3505\"}]},\"type\":\"ConnectorPlacement.EquallySpacedConnector\",\"uuid\":\"c80211c6-bb24-481b-97ca-2752015f3b18\"}],\"packageUris\":[\"http://schema.mathworks.com/mf0/Connector/19700101\"],\"version\":\"1.0\"}"
  Tile122 : Subsystem  mask(Square Tile){side=side, thickness=thick, color=color2, opacity=opacity}
      mask prompts: side "Side (m) :"; thickness "Thickness (m) :"; color "Color [RGB] :"; opacity "Opacity (0...1) :"
      mask help: This block creates a flat, single, square tile element. The square tile body is mass-less, so it will not have an effect on the dynamic simulation. This square tile element can be used as a graphic reference by itself, or as part of a composite graphic reference made of an array of interconnected tiles. The square tile is aligned with the XY plane, and the block provides frame connector ports to the middle points on each of the four sides of the body of the square - right (+X), left (-X), top (+Y) and bottom (-Y). All dimensions are in meters.
      settings: PortSchema="{\"entries\":[{\"content\":{\"sides\":[{\"content\":{\"connectorIds\":[\"LConn1\"]},\"type\":\"ConnectorPlacement.EquallySpacedRectSide\",\"uuid\":\"a971723f-ea37-4e9b-910b-501b94fb0ba2\"},{\"content\":{\"connectorIds\":[\"RConn1\"],\"side\":\"RIGHT\"},\"type\":\"ConnectorPlacement.EquallySpacedRectSide\",\"uuid\":\"e50175c1-005c-4b0b-bced-b882197eaab2\"},{\"content\":{\"connectorIds\":[\"LConn2\"],\"side\":\"TOP\"},\"type\":\"ConnectorPlacement.EquallySpacedRectSide\",\"uuid\":\"2a04a964-d53e-47ee-8c79-d53dd599bafe\"},{\"content\":{\"connectorIds\":[\"RConn2\"],\"side\":\"BOTTOM\"},\"type\":\"ConnectorPlacement.EquallySpacedRectSide\",\"uuid\":\"a0066dd6-a193-491c-afbe-bac00dfc3505\"}]},\"type\":\"ConnectorPlacement.EquallySpacedConnector\",\"uuid\":\"c80211c6-bb24-481b-97ca-2752015f3b18\"}],\"packageUris\":[\"http://schema.mathworks.com/mf0/Connector/19700101\"],\"version\":\"1.0\"}"
  Tile123 : Subsystem  mask(Square Tile){side=side, thickness=thick, color=color1, opacity=opacity}
      mask prompts: side "Side (m) :"; thickness "Thickness (m) :"; color "Color [RGB] :"; opacity "Opacity (0...1) :"
      mask help: This block creates a flat, single, square tile element. The square tile body is mass-less, so it will not have an effect on the dynamic simulation. This square tile element can be used as a graphic reference by itself, or as part of a composite graphic reference made of an array of interconnected tiles. The square tile is aligned with the XY plane, and the block provides frame connector ports to the middle points on each of the four sides of the body of the square - right (+X), left (-X), top (+Y) and bottom (-Y). All dimensions are in meters.
      settings: PortSchema="{\"entries\":[{\"content\":{\"sides\":[{\"content\":{\"connectorIds\":[\"LConn1\"]},\"type\":\"ConnectorPlacement.EquallySpacedRectSide\",\"uuid\":\"a971723f-ea37-4e9b-910b-501b94fb0ba2\"},{\"content\":{\"connectorIds\":[\"RConn1\"],\"side\":\"RIGHT\"},\"type\":\"ConnectorPlacement.EquallySpacedRectSide\",\"uuid\":\"e50175c1-005c-4b0b-bced-b882197eaab2\"},{\"content\":{\"connectorIds\":[\"LConn2\"],\"side\":\"TOP\"},\"type\":\"ConnectorPlacement.EquallySpacedRectSide\",\"uuid\":\"2a04a964-d53e-47ee-8c79-d53dd599bafe\"},{\"content\":{\"connectorIds\":[\"RConn2\"],\"side\":\"BOTTOM\"},\"type\":\"ConnectorPlacement.EquallySpacedRectSide\",\"uuid\":\"a0066dd6-a193-491c-afbe-bac00dfc3505\"}]},\"type\":\"ConnectorPlacement.EquallySpacedConnector\",\"uuid\":\"c80211c6-bb24-481b-97ca-2752015f3b18\"}],\"packageUris\":[\"http://schema.mathworks.com/mf0/Connector/19700101\"],\"version\":\"1.0\"}"
  Tile124 : Subsystem  mask(Square Tile){side=side, thickness=thick, color=color2, opacity=opacity}
      mask prompts: side "Side (m) :"; thickness "Thickness (m) :"; color "Color [RGB] :"; opacity "Opacity (0...1) :"
      mask help: This block creates a flat, single, square tile element. The square tile body is mass-less, so it will not have an effect on the dynamic simulation. This square tile element can be used as a graphic reference by itself, or as part of a composite graphic reference made of an array of interconnected tiles. The square tile is aligned with the XY plane, and the block provides frame connector ports to the middle points on each of the four sides of the body of the square - right (+X), left (-X), top (+Y) and bottom (-Y). All dimensions are in meters.
      settings: PortSchema="{\"entries\":[{\"content\":{\"sides\":[{\"content\":{\"connectorIds\":[\"LConn1\"]},\"type\":\"ConnectorPlacement.EquallySpacedRectSide\",\"uuid\":\"a971723f-ea37-4e9b-910b-501b94fb0ba2\"},{\"content\":{\"connectorIds\":[\"RConn1\"],\"side\":\"RIGHT\"},\"type\":\"ConnectorPlacement.EquallySpacedRectSide\",\"uuid\":\"e50175c1-005c-4b0b-bced-b882197eaab2\"},{\"content\":{\"connectorIds\":[\"LConn2\"],\"side\":\"TOP\"},\"type\":\"ConnectorPlacement.EquallySpacedRectSide\",\"uuid\":\"2a04a964-d53e-47ee-8c79-d53dd599bafe\"},{\"content\":{\"connectorIds\":[\"RConn2\"],\"side\":\"BOTTOM\"},\"type\":\"ConnectorPlacement.EquallySpacedRectSide\",\"uuid\":\"a0066dd6-a193-491c-afbe-bac00dfc3505\"}]},\"type\":\"ConnectorPlacement.EquallySpacedConnector\",\"uuid\":\"c80211c6-bb24-481b-97ca-2752015f3b18\"}],\"packageUris\":[\"http://schema.mathworks.com/mf0/Connector/19700101\"],\"version\":\"1.0\"}"
  Tile125 : Subsystem  mask(Square Tile){side=side, thickness=thick, color=color1, opacity=opacity}
      mask prompts: side "Side (m) :"; thickness "Thickness (m) :"; color "Color [RGB] :"; opacity "Opacity (0...1) :"
      mask help: This block creates a flat, single, square tile element. The square tile body is mass-less, so it will not have an effect on the dynamic simulation. This square tile element can be used as a graphic reference by itself, or as part of a composite graphic reference made of an array of interconnected tiles. The square tile is aligned with the XY plane, and the block provides frame connector ports to the middle points on each of the four sides of the body of the square - right (+X), left (-X), top (+Y) and bottom (-Y). All dimensions are in meters.
      settings: PortSchema="{\"entries\":[{\"content\":{\"sides\":[{\"content\":{\"connectorIds\":[\"LConn1\"]},\"type\":\"ConnectorPlacement.EquallySpacedRectSide\",\"uuid\":\"a971723f-ea37-4e9b-910b-501b94fb0ba2\"},{\"content\":{\"connectorIds\":[\"RConn1\"],\"side\":\"RIGHT\"},\"type\":\"ConnectorPlacement.EquallySpacedRectSide\",\"uuid\":\"e50175c1-005c-4b0b-bced-b882197eaab2\"},{\"content\":{\"connectorIds\":[\"LConn2\"],\"side\":\"TOP\"},\"type\":\"ConnectorPlacement.EquallySpacedRectSide\",\"uuid\":\"2a04a964-d53e-47ee-8c79-d53dd599bafe\"},{\"content\":{\"connectorIds\":[\"RConn2\"],\"side\":\"BOTTOM\"},\"type\":\"ConnectorPlacement.EquallySpacedRectSide\",\"uuid\":\"a0066dd6-a193-491c-afbe-bac00dfc3505\"}]},\"type\":\"ConnectorPlacement.EquallySpacedConnector\",\"uuid\":\"c80211c6-bb24-481b-97ca-2752015f3b18\"}],\"packageUris\":[\"http://schema.mathworks.com/mf0/Connector/19700101\"],\"version\":\"1.0\"}"
  Tile126 : Subsystem  mask(Square Tile){side=side, thickness=thick, color=color2, opacity=opacity}
      mask prompts: side "Side (m) :"; thickness "Thickness (m) :"; color "Color [RGB] :"; opacity "Opacity (0...1) :"
      mask help: This block creates a flat, single, square tile element. The square tile body is mass-less, so it will not have an effect on the dynamic simulation. This square tile element can be used as a graphic reference by itself, or as part of a composite graphic reference made of an array of interconnected tiles. The square tile is aligned with the XY plane, and the block provides frame connector ports to the middle points on each of the four sides of the body of the square - right (+X), left (-X), top (+Y) and bottom (-Y). All dimensions are in meters.
      settings: PortSchema="{\"entries\":[{\"content\":{\"sides\":[{\"content\":{\"connectorIds\":[\"LConn1\"]},\"type\":\"ConnectorPlacement.EquallySpacedRectSide\",\"uuid\":\"a971723f-ea37-4e9b-910b-501b94fb0ba2\"},{\"content\":{\"connectorIds\":[\"RConn1\"],\"side\":\"RIGHT\"},\"type\":\"ConnectorPlacement.EquallySpacedRectSide\",\"uuid\":\"e50175c1-005c-4b0b-bced-b882197eaab2\"},{\"content\":{\"connectorIds\":[\"LConn2\"],\"side\":\"TOP\"},\"type\":\"ConnectorPlacement.EquallySpacedRectSide\",\"uuid\":\"2a04a964-d53e-47ee-8c79-d53dd599bafe\"},{\"content\":{\"connectorIds\":[\"RConn2\"],\"side\":\"BOTTOM\"},\"type\":\"ConnectorPlacement.EquallySpacedRectSide\",\"uuid\":\"a0066dd6-a193-491c-afbe-bac00dfc3505\"}]},\"type\":\"ConnectorPlacement.EquallySpacedConnector\",\"uuid\":\"c80211c6-bb24-481b-97ca-2752015f3b18\"}],\"packageUris\":[\"http://schema.mathworks.com/mf0/Connector/19700101\"],\"version\":\"1.0\"}"
  Tile127 : Subsystem  mask(Square Tile){side=side, thickness=thick, color=color1, opacity=opacity}
      mask prompts: side "Side (m) :"; thickness "Thickness (m) :"; color "Color [RGB] :"; opacity "Opacity (0...1) :"
      mask help: This block creates a flat, single, square tile element. The square tile body is mass-less, so it will not have an effect on the dynamic simulation. This square tile element can be used as a graphic reference by itself, or as part of a composite graphic reference made of an array of interconnected tiles. The square tile is aligned with the XY plane, and the block provides frame connector ports to the middle points on each of the four sides of the body of the square - right (+X), left (-X), top (+Y) and bottom (-Y). All dimensions are in meters.
      settings: PortSchema="{\"entries\":[{\"content\":{\"sides\":[{\"content\":{\"connectorIds\":[\"LConn1\"]},\"type\":\"ConnectorPlacement.EquallySpacedRectSide\",\"uuid\":\"a971723f-ea37-4e9b-910b-501b94fb0ba2\"},{\"content\":{\"connectorIds\":[\"RConn1\"],\"side\":\"RIGHT\"},\"type\":\"ConnectorPlacement.EquallySpacedRectSide\",\"uuid\":\"e50175c1-005c-4b0b-bced-b882197eaab2\"},{\"content\":{\"connectorIds\":[\"LConn2\"],\"side\":\"TOP\"},\"type\":\"ConnectorPlacement.EquallySpacedRectSide\",\"uuid\":\"2a04a964-d53e-47ee-8c79-d53dd599bafe\"},{\"content\":{\"connectorIds\":[\"RConn2\"],\"side\":\"BOTTOM\"},\"type\":\"ConnectorPlacement.EquallySpacedRectSide\",\"uuid\":\"a0066dd6-a193-491c-afbe-bac00dfc3505\"}]},\"type\":\"ConnectorPlacement.EquallySpacedConnector\",\"uuid\":\"c80211c6-bb24-481b-97ca-2752015f3b18\"}],\"packageUris\":[\"http://schema.mathworks.com/mf0/Connector/19700101\"],\"version\":\"1.0\"}"
  Tile128 : Subsystem  mask(Square Tile){side=side, thickness=thick, color=color1, opacity=opacity}
      mask prompts: side "Side (m) :"; thickness "Thickness (m) :"; color "Color [RGB] :"; opacity "Opacity (0...1) :"
      mask help: This block creates a flat, single, square tile element. The square tile body is mass-less, so it will not have an effect on the dynamic simulation. This square tile element can be used as a graphic reference by itself, or as part of a composite graphic reference made of an array of interconnected tiles. The square tile is aligned with the XY plane, and the block provides frame connector ports to the middle points on each of the four sides of the body of the square - right (+X), left (-X), top (+Y) and bottom (-Y). All dimensions are in meters.
      settings: PortSchema="{\"entries\":[{\"content\":{\"sides\":[{\"content\":{\"connectorIds\":[\"LConn1\"]},\"type\":\"ConnectorPlacement.EquallySpacedRectSide\",\"uuid\":\"a971723f-ea37-4e9b-910b-501b94fb0ba2\"},{\"content\":{\"connectorIds\":[\"RConn1\"],\"side\":\"RIGHT\"},\"type\":\"ConnectorPlacement.EquallySpacedRectSide\",\"uuid\":\"e50175c1-005c-4b0b-bced-b882197eaab2\"},{\"content\":{\"connectorIds\":[\"LConn2\"],\"side\":\"TOP\"},\"type\":\"ConnectorPlacement.EquallySpacedRectSide\",\"uuid\":\"2a04a964-d53e-47ee-8c79-d53dd599bafe\"},{\"content\":{\"connectorIds\":[\"RConn2\"],\"side\":\"BOTTOM\"},\"type\":\"ConnectorPlacement.EquallySpacedRectSide\",\"uuid\":\"a0066dd6-a193-491c-afbe-bac00dfc3505\"}]},\"type\":\"ConnectorPlacement.EquallySpacedConnector\",\"uuid\":\"c80211c6-bb24-481b-97ca-2752015f3b18\"}],\"packageUris\":[\"http://schema.mathworks.com/mf0/Connector/19700101\"],\"version\":\"1.0\"}"
  Tile129 : Subsystem  mask(Square Tile){side=side, thickness=thick, color=color2, opacity=opacity}
      mask prompts: side "Side (m) :"; thickness "Thickness (m) :"; color "Color [RGB] :"; opacity "Opacity (0...1) :"
      mask help: This block creates a flat, single, square tile element. The square tile body is mass-less, so it will not have an effect on the dynamic simulation. This square tile element can be used as a graphic reference by itself, or as part of a composite graphic reference made of an array of interconnected tiles. The square tile is aligned with the XY plane, and the block provides frame connector ports to the middle points on each of the four sides of the body of the square - right (+X), left (-X), top (+Y) and bottom (-Y). All dimensions are in meters.
      settings: PortSchema="{\"entries\":[{\"content\":{\"sides\":[{\"content\":{\"connectorIds\":[\"LConn1\"]},\"type\":\"ConnectorPlacement.EquallySpacedRectSide\",\"uuid\":\"a971723f-ea37-4e9b-910b-501b94fb0ba2\"},{\"content\":{\"connectorIds\":[\"RConn1\"],\"side\":\"RIGHT\"},\"type\":\"ConnectorPlacement.EquallySpacedRectSide\",\"uuid\":\"e50175c1-005c-4b0b-bced-b882197eaab2\"},{\"content\":{\"connectorIds\":[\"LConn2\"],\"side\":\"TOP\"},\"type\":\"ConnectorPlacement.EquallySpacedRectSide\",\"uuid\":\"2a04a964-d53e-47ee-8c79-d53dd599bafe\"},{\"content\":{\"connectorIds\":[\"RConn2\"],\"side\":\"BOTTOM\"},\"type\":\"ConnectorPlacement.EquallySpacedRectSide\",\"uuid\":\"a0066dd6-a193-491c-afbe-bac00dfc3505\"}]},\"type\":\"ConnectorPlacement.EquallySpacedConnector\",\"uuid\":\"c80211c6-bb24-481b-97ca-2752015f3b18\"}],\"packageUris\":[\"http://schema.mathworks.com/mf0/Connector/19700101\"],\"version\":\"1.0\"}"
  Tile13 : Subsystem  mask(Square Tile){side=side, thickness=thick, color=color1, opacity=opacity}
      mask prompts: side "Side (m) :"; thickness "Thickness (m) :"; color "Color [RGB] :"; opacity "Opacity (0...1) :"
      mask help: This block creates a flat, single, square tile element. The square tile body is mass-less, so it will not have an effect on the dynamic simulation. This square tile element can be used as a graphic reference by itself, or as part of a composite graphic reference made of an array of interconnected tiles. The square tile is aligned with the XY plane, and the block provides frame connector ports to the middle points on each of the four sides of the body of the square - right (+X), left (-X), top (+Y) and bottom (-Y). All dimensions are in meters.
      settings: PortSchema="{\"entries\":[{\"content\":{\"sides\":[{\"content\":{\"connectorIds\":[\"LConn1\"]},\"type\":\"ConnectorPlacement.EquallySpacedRectSide\",\"uuid\":\"a971723f-ea37-4e9b-910b-501b94fb0ba2\"},{\"content\":{\"connectorIds\":[\"RConn1\"],\"side\":\"RIGHT\"},\"type\":\"ConnectorPlacement.EquallySpacedRectSide\",\"uuid\":\"e50175c1-005c-4b0b-bced-b882197eaab2\"},{\"content\":{\"connectorIds\":[\"LConn2\"],\"side\":\"TOP\"},\"type\":\"ConnectorPlacement.EquallySpacedRectSide\",\"uuid\":\"2a04a964-d53e-47ee-8c79-d53dd599bafe\"},{\"content\":{\"connectorIds\":[\"RConn2\"],\"side\":\"BOTTOM\"},\"type\":\"ConnectorPlacement.EquallySpacedRectSide\",\"uuid\":\"a0066dd6-a193-491c-afbe-bac00dfc3505\"}]},\"type\":\"ConnectorPlacement.EquallySpacedConnector\",\"uuid\":\"c80211c6-bb24-481b-97ca-2752015f3b18\"}],\"packageUris\":[\"http://schema.mathworks.com/mf0/Connector/19700101\"],\"version\":\"1.0\"}"
  Tile130 : Subsystem  mask(Square Tile){side=side, thickness=thick, color=color2, opacity=opacity}
      mask prompts: side "Side (m) :"; thickness "Thickness (m) :"; color "Color [RGB] :"; opacity "Opacity (0...1) :"
      mask help: This block creates a flat, single, square tile element. The square tile body is mass-less, so it will not have an effect on the dynamic simulation. This square tile element can be used as a graphic reference by itself, or as part of a composite graphic reference made of an array of interconnected tiles. The square tile is aligned with the XY plane, and the block provides frame connector ports to the middle points on each of the four sides of the body of the square - right (+X), left (-X), top (+Y) and bottom (-Y). All dimensions are in meters.
      settings: PortSchema="{\"entries\":[{\"content\":{\"sides\":[{\"content\":{\"connectorIds\":[\"LConn1\"]},\"type\":\"ConnectorPlacement.EquallySpacedRectSide\",\"uuid\":\"a971723f-ea37-4e9b-910b-501b94fb0ba2\"},{\"content\":{\"connectorIds\":[\"RConn1\"],\"side\":\"RIGHT\"},\"type\":\"ConnectorPlacement.EquallySpacedRectSide\",\"uuid\":\"e50175c1-005c-4b0b-bced-b882197eaab2\"},{\"content\":{\"connectorIds\":[\"LConn2\"],\"side\":\"TOP\"},\"type\":\"ConnectorPlacement.EquallySpacedRectSide\",\"uuid\":\"2a04a964-d53e-47ee-8c79-d53dd599bafe\"},{\"content\":{\"connectorIds\":[\"RConn2\"],\"side\":\"BOTTOM\"},\"type\":\"ConnectorPlacement.EquallySpacedRectSide\",\"uuid\":\"a0066dd6-a193-491c-afbe-bac00dfc3505\"}]},\"type\":\"ConnectorPlacement.EquallySpacedConnector\",\"uuid\":\"c80211c6-bb24-481b-97ca-2752015f3b18\"}],\"packageUris\":[\"http://schema.mathworks.com/mf0/Connector/19700101\"],\"version\":\"1.0\"}"
  Tile131 : Subsystem  mask(Square Tile){side=side, thickness=thick, color=color2, opacity=opacity}
      mask prompts: side "Side (m) :"; thickness "Thickness (m) :"; color "Color [RGB] :"; opacity "Opacity (0...1) :"
      mask help: This block creates a flat, single, square tile element. The square tile body is mass-less, so it will not have an effect on the dynamic simulation. This square tile element can be used as a graphic reference by itself, or as part of a composite graphic reference made of an array of interconnected tiles. The square tile is aligned with the XY plane, and the block provides frame connector ports to the middle points on each of the four sides of the body of the square - right (+X), left (-X), top (+Y) and bottom (-Y). All dimensions are in meters.
      settings: PortSchema="{\"entries\":[{\"content\":{\"sides\":[{\"content\":{\"connectorIds\":[\"LConn1\"]},\"type\":\"ConnectorPlacement.EquallySpacedRectSide\",\"uuid\":\"a971723f-ea37-4e9b-910b-501b94fb0ba2\"},{\"content\":{\"connectorIds\":[\"RConn1\"],\"side\":\"RIGHT\"},\"type\":\"ConnectorPlacement.EquallySpacedRectSide\",\"uuid\":\"e50175c1-005c-4b0b-bced-b882197eaab2\"},{\"content\":{\"connectorIds\":[\"LConn2\"],\"side\":\"TOP\"},\"type\":\"ConnectorPlacement.EquallySpacedRectSide\",\"uuid\":\"2a04a964-d53e-47ee-8c79-d53dd599bafe\"},{\"content\":{\"connectorIds\":[\"RConn2\"],\"side\":\"BOTTOM\"},\"type\":\"ConnectorPlacement.EquallySpacedRectSide\",\"uuid\":\"a0066dd6-a193-491c-afbe-bac00dfc3505\"}]},\"type\":\"ConnectorPlacement.EquallySpacedConnector\",\"uuid\":\"c80211c6-bb24-481b-97ca-2752015f3b18\"}],\"packageUris\":[\"http://schema.mathworks.com/mf0/Connector/19700101\"],\"version\":\"1.0\"}"
  Tile132 : Subsystem  mask(Square Tile){side=side, thickness=thick, color=color1, opacity=opacity}
      mask prompts: side "Side (m) :"; thickness "Thickness (m) :"; color "Color [RGB] :"; opacity "Opacity (0...1) :"
      mask help: This block creates a flat, single, square tile element. The square tile body is mass-less, so it will not have an effect on the dynamic simulation. This square tile element can be used as a graphic reference by itself, or as part of a composite graphic reference made of an array of interconnected tiles. The square tile is aligned with the XY plane, and the block provides frame connector ports to the middle points on each of the four sides of the body of the square - right (+X), left (-X), top (+Y) and bottom (-Y). All dimensions are in meters.
      settings: PortSchema="{\"entries\":[{\"content\":{\"sides\":[{\"content\":{\"connectorIds\":[\"LConn1\"]},\"type\":\"ConnectorPlacement.EquallySpacedRectSide\",\"uuid\":\"a971723f-ea37-4e9b-910b-501b94fb0ba2\"},{\"content\":{\"connectorIds\":[\"RConn1\"],\"side\":\"RIGHT\"},\"type\":\"ConnectorPlacement.EquallySpacedRectSide\",\"uuid\":\"e50175c1-005c-4b0b-bced-b882197eaab2\"},{\"content\":{\"connectorIds\":[\"LConn2\"],\"side\":\"TOP\"},\"type\":\"ConnectorPlacement.EquallySpacedRectSide\",\"uuid\":\"2a04a964-d53e-47ee-8c79-d53dd599bafe\"},{\"content\":{\"connectorIds\":[\"RConn2\"],\"side\":\"BOTTOM\"},\"type\":\"ConnectorPlacement.EquallySpacedRectSide\",\"uuid\":\"a0066dd6-a193-491c-afbe-bac00dfc3505\"}]},\"type\":\"ConnectorPlacement.EquallySpacedConnector\",\"uuid\":\"c80211c6-bb24-481b-97ca-2752015f3b18\"}],\"packageUris\":[\"http://schema.mathworks.com/mf0/Connector/19700101\"],\"version\":\"1.0\"}"
  Tile133 : Subsystem  mask(Square Tile){side=side, thickness=thick, color=color1, opacity=opacity}
      mask prompts: side "Side (m) :"; thickness "Thickness (m) :"; color "Color [RGB] :"; opacity "Opacity (0...1) :"
      mask help: This block creates a flat, single, square tile element. The square tile body is mass-less, so it will not have an effect on the dynamic simulation. This square tile element can be used as a graphic reference by itself, or as part of a composite graphic reference made of an array of interconnected tiles. The square tile is aligned with the XY plane, and the block provides frame connector ports to the middle points on each of the four sides of the body of the square - right (+X), left (-X), top (+Y) and bottom (-Y). All dimensions are in meters.
      settings: PortSchema="{\"entries\":[{\"content\":{\"sides\":[{\"content\":{\"connectorIds\":[\"LConn1\"]},\"type\":\"ConnectorPlacement.EquallySpacedRectSide\",\"uuid\":\"a971723f-ea37-4e9b-910b-501b94fb0ba2\"},{\"content\":{\"connectorIds\":[\"RConn1\"],\"side\":\"RIGHT\"},\"type\":\"ConnectorPlacement.EquallySpacedRectSide\",\"uuid\":\"e50175c1-005c-4b0b-bced-b882197eaab2\"},{\"content\":{\"connectorIds\":[\"LConn2\"],\"side\":\"TOP\"},\"type\":\"ConnectorPlacement.EquallySpacedRectSide\",\"uuid\":\"2a04a964-d53e-47ee-8c79-d53dd599bafe\"},{\"content\":{\"connectorIds\":[\"RConn2\"],\"side\":\"BOTTOM\"},\"type\":\"ConnectorPlacement.EquallySpacedRectSide\",\"uuid\":\"a0066dd6-a193-491c-afbe-bac00dfc3505\"}]},\"type\":\"ConnectorPlacement.EquallySpacedConnector\",\"uuid\":\"c80211c6-bb24-481b-97ca-2752015f3b18\"}],\"packageUris\":[\"http://schema.mathworks.com/mf0/Connector/19700101\"],\"version\":\"1.0\"}"
  Tile134 : Subsystem  mask(Square Tile){side=side, thickness=thick, color=color2, opacity=opacity}
      mask prompts: side "Side (m) :"; thickness "Thickness (m) :"; color "Color [RGB] :"; opacity "Opacity (0...1) :"
      mask help: This block creates a flat, single, square tile element. The square tile body is mass-less, so it will not have an effect on the dynamic simulation. This square tile element can be used as a graphic reference by itself, or as part of a composite graphic reference made of an array of interconnected tiles. The square tile is aligned with the XY plane, and the block provides frame connector ports to the middle points on each of the four sides of the body of the square - right (+X), left (-X), top (+Y) and bottom (-Y). All dimensions are in meters.
      settings: PortSchema="{\"entries\":[{\"content\":{\"sides\":[{\"content\":{\"connectorIds\":[\"LConn1\"]},\"type\":\"ConnectorPlacement.EquallySpacedRectSide\",\"uuid\":\"a971723f-ea37-4e9b-910b-501b94fb0ba2\"},{\"content\":{\"connectorIds\":[\"RConn1\"],\"side\":\"RIGHT\"},\"type\":\"ConnectorPlacement.EquallySpacedRectSide\",\"uuid\":\"e50175c1-005c-4b0b-bced-b882197eaab2\"},{\"content\":{\"connectorIds\":[\"LConn2\"],\"side\":\"TOP\"},\"type\":\"ConnectorPlacement.EquallySpacedRectSide\",\"uuid\":\"2a04a964-d53e-47ee-8c79-d53dd599bafe\"},{\"content\":{\"connectorIds\":[\"RConn2\"],\"side\":\"BOTTOM\"},\"type\":\"ConnectorPlacement.EquallySpacedRectSide\",\"uuid\":\"a0066dd6-a193-491c-afbe-bac00dfc3505\"}]},\"type\":\"ConnectorPlacement.EquallySpacedConnector\",\"uuid\":\"c80211c6-bb24-481b-97ca-2752015f3b18\"}],\"packageUris\":[\"http://schema.mathworks.com/mf0/Connector/19700101\"],\"version\":\"1.0\"}"
  Tile135 : Subsystem  mask(Square Tile){side=side, thickness=thick, color=color2, opacity=opacity}
      mask prompts: side "Side (m) :"; thickness "Thickness (m) :"; color "Color [RGB] :"; opacity "Opacity (0...1) :"
      mask help: This block creates a flat, single, square tile element. The square tile body is mass-less, so it will not have an effect on the dynamic simulation. This square tile element can be used as a graphic reference by itself, or as part of a composite graphic reference made of an array of interconnected tiles. The square tile is aligned with the XY plane, and the block provides frame connector ports to the middle points on each of the four sides of the body of the square - right (+X), left (-X), top (+Y) and bottom (-Y). All dimensions are in meters.
      settings: PortSchema="{\"entries\":[{\"content\":{\"sides\":[{\"content\":{\"connectorIds\":[\"LConn1\"]},\"type\":\"ConnectorPlacement.EquallySpacedRectSide\",\"uuid\":\"a971723f-ea37-4e9b-910b-501b94fb0ba2\"},{\"content\":{\"connectorIds\":[\"RConn1\"],\"side\":\"RIGHT\"},\"type\":\"ConnectorPlacement.EquallySpacedRectSide\",\"uuid\":\"e50175c1-005c-4b0b-bced-b882197eaab2\"},{\"content\":{\"connectorIds\":[\"LConn2\"],\"side\":\"TOP\"},\"type\":\"ConnectorPlacement.EquallySpacedRectSide\",\"uuid\":\"2a04a964-d53e-47ee-8c79-d53dd599bafe\"},{\"content\":{\"connectorIds\":[\"RConn2\"],\"side\":\"BOTTOM\"},\"type\":\"ConnectorPlacement.EquallySpacedRectSide\",\"uuid\":\"a0066dd6-a193-491c-afbe-bac00dfc3505\"}]},\"type\":\"ConnectorPlacement.EquallySpacedConnector\",\"uuid\":\"c80211c6-bb24-481b-97ca-2752015f3b18\"}],\"packageUris\":[\"http://schema.mathworks.com/mf0/Connector/19700101\"],\"version\":\"1.0\"}"
  Tile136 : Subsystem  mask(Square Tile){side=side, thickness=thick, color=color2, opacity=opacity}
      mask prompts: side "Side (m) :"; thickness "Thickness (m) :"; color "Color [RGB] :"; opacity "Opacity (0...1) :"
      mask help: This block creates a flat, single, square tile element. The square tile body is mass-less, so it will not have an effect on the dynamic simulation. This square tile element can be used as a graphic reference by itself, or as part of a composite graphic reference made of an array of interconnected tiles. The square tile is aligned with the XY plane, and the block provides frame connector ports to the middle points on each of the four sides of the body of the square - right (+X), left (-X), top (+Y) and bottom (-Y). All dimensions are in meters.
      settings: PortSchema="{\"entries\":[{\"content\":{\"sides\":[{\"content\":{\"connectorIds\":[\"LConn1\"]},\"type\":\"ConnectorPlacement.EquallySpacedRectSide\",\"uuid\":\"a971723f-ea37-4e9b-910b-501b94fb0ba2\"},{\"content\":{\"connectorIds\":[\"RConn1\"],\"side\":\"RIGHT\"},\"type\":\"ConnectorPlacement.EquallySpacedRectSide\",\"uuid\":\"e50175c1-005c-4b0b-bced-b882197eaab2\"},{\"content\":{\"connectorIds\":[\"LConn2\"],\"side\":\"TOP\"},\"type\":\"ConnectorPlacement.EquallySpacedRectSide\",\"uuid\":\"2a04a964-d53e-47ee-8c79-d53dd599bafe\"},{\"content\":{\"connectorIds\":[\"RConn2\"],\"side\":\"BOTTOM\"},\"type\":\"ConnectorPlacement.EquallySpacedRectSide\",\"uuid\":\"a0066dd6-a193-491c-afbe-bac00dfc3505\"}]},\"type\":\"ConnectorPlacement.EquallySpacedConnector\",\"uuid\":\"c80211c6-bb24-481b-97ca-2752015f3b18\"}],\"packageUris\":[\"http://schema.mathworks.com/mf0/Connector/19700101\"],\"version\":\"1.0\"}"
  Tile137 : Subsystem  mask(Square Tile){side=side, thickness=thick, color=color1, opacity=opacity}
      mask prompts: side "Side (m) :"; thickness "Thickness (m) :"; color "Color [RGB] :"; opacity "Opacity (0...1) :"
      mask help: This block creates a flat, single, square tile element. The square tile body is mass-less, so it will not have an effect on the dynamic simulation. This square tile element can be used as a graphic reference by itself, or as part of a composite graphic reference made of an array of interconnected tiles. The square tile is aligned with the XY plane, and the block provides frame connector ports to the middle points on each of the four sides of the body of the square - right (+X), left (-X), top (+Y) and bottom (-Y). All dimensions are in meters.
      settings: PortSchema="{\"entries\":[{\"content\":{\"sides\":[{\"content\":{\"connectorIds\":[\"LConn1\"]},\"type\":\"ConnectorPlacement.EquallySpacedRectSide\",\"uuid\":\"a971723f-ea37-4e9b-910b-501b94fb0ba2\"},{\"content\":{\"connectorIds\":[\"RConn1\"],\"side\":\"RIGHT\"},\"type\":\"ConnectorPlacement.EquallySpacedRectSide\",\"uuid\":\"e50175c1-005c-4b0b-bced-b882197eaab2\"},{\"content\":{\"connectorIds\":[\"LConn2\"],\"side\":\"TOP\"},\"type\":\"ConnectorPlacement.EquallySpacedRectSide\",\"uuid\":\"2a04a964-d53e-47ee-8c79-d53dd599bafe\"},{\"content\":{\"connectorIds\":[\"RConn2\"],\"side\":\"BOTTOM\"},\"type\":\"ConnectorPlacement.EquallySpacedRectSide\",\"uuid\":\"a0066dd6-a193-491c-afbe-bac00dfc3505\"}]},\"type\":\"ConnectorPlacement.EquallySpacedConnector\",\"uuid\":\"c80211c6-bb24-481b-97ca-2752015f3b18\"}],\"packageUris\":[\"http://schema.mathworks.com/mf0/Connector/19700101\"],\"version\":\"1.0\"}"
  Tile138 : Subsystem  mask(Square Tile){side=side, thickness=thick, color=color1, opacity=opacity}
      mask prompts: side "Side (m) :"; thickness "Thickness (m) :"; color "Color [RGB] :"; opacity "Opacity (0...1) :"
      mask help: This block creates a flat, single, square tile element. The square tile body is mass-less, so it will not have an effect on the dynamic simulation. This square tile element can be used as a graphic reference by itself, or as part of a composite graphic reference made of an array of interconnected tiles. The square tile is aligned with the XY plane, and the block provides frame connector ports to the middle points on each of the four sides of the body of the square - right (+X), left (-X), top (+Y) and bottom (-Y). All dimensions are in meters.
      settings: PortSchema="{\"entries\":[{\"content\":{\"sides\":[{\"content\":{\"connectorIds\":[\"LConn1\"]},\"type\":\"ConnectorPlacement.EquallySpacedRectSide\",\"uuid\":\"a971723f-ea37-4e9b-910b-501b94fb0ba2\"},{\"content\":{\"connectorIds\":[\"RConn1\"],\"side\":\"RIGHT\"},\"type\":\"ConnectorPlacement.EquallySpacedRectSide\",\"uuid\":\"e50175c1-005c-4b0b-bced-b882197eaab2\"},{\"content\":{\"connectorIds\":[\"LConn2\"],\"side\":\"TOP\"},\"type\":\"ConnectorPlacement.EquallySpacedRectSide\",\"uuid\":\"2a04a964-d53e-47ee-8c79-d53dd599bafe\"},{\"content\":{\"connectorIds\":[\"RConn2\"],\"side\":\"BOTTOM\"},\"type\":\"ConnectorPlacement.EquallySpacedRectSide\",\"uuid\":\"a0066dd6-a193-491c-afbe-bac00dfc3505\"}]},\"type\":\"ConnectorPlacement.EquallySpacedConnector\",\"uuid\":\"c80211c6-bb24-481b-97ca-2752015f3b18\"}],\"packageUris\":[\"http://schema.mathworks.com/mf0/Connector/19700101\"],\"version\":\"1.0\"}"
  Tile139 : Subsystem  mask(Square Tile){side=side, thickness=thick, color=color1, opacity=opacity}
      mask prompts: side "Side (m) :"; thickness "Thickness (m) :"; color "Color [RGB] :"; opacity "Opacity (0...1) :"
      mask help: This block creates a flat, single, square tile element. The square tile body is mass-less, so it will not have an effect on the dynamic simulation. This square tile element can be used as a graphic reference by itself, or as part of a composite graphic reference made of an array of interconnected tiles. The square tile is aligned with the XY plane, and the block provides frame connector ports to the middle points on each of the four sides of the body of the square - right (+X), left (-X), top (+Y) and bottom (-Y). All dimensions are in meters.
      settings: PortSchema="{\"entries\":[{\"content\":{\"sides\":[{\"content\":{\"connectorIds\":[\"LConn1\"]},\"type\":\"ConnectorPlacement.EquallySpacedRectSide\",\"uuid\":\"a971723f-ea37-4e9b-910b-501b94fb0ba2\"},{\"content\":{\"connectorIds\":[\"RConn1\"],\"side\":\"RIGHT\"},\"type\":\"ConnectorPlacement.EquallySpacedRectSide\",\"uuid\":\"e50175c1-005c-4b0b-bced-b882197eaab2\"},{\"content\":{\"connectorIds\":[\"LConn2\"],\"side\":\"TOP\"},\"type\":\"ConnectorPlacement.EquallySpacedRectSide\",\"uuid\":\"2a04a964-d53e-47ee-8c79-d53dd599bafe\"},{\"content\":{\"connectorIds\":[\"RConn2\"],\"side\":\"BOTTOM\"},\"type\":\"ConnectorPlacement.EquallySpacedRectSide\",\"uuid\":\"a0066dd6-a193-491c-afbe-bac00dfc3505\"}]},\"type\":\"ConnectorPlacement.EquallySpacedConnector\",\"uuid\":\"c80211c6-bb24-481b-97ca-2752015f3b18\"}],\"packageUris\":[\"http://schema.mathworks.com/mf0/Connector/19700101\"],\"version\":\"1.0\"}"
  Tile14 : Subsystem  mask(Square Tile){side=side, thickness=thick, color=color2, opacity=opacity}
      mask prompts: side "Side (m) :"; thickness "Thickness (m) :"; color "Color [RGB] :"; opacity "Opacity (0...1) :"
      mask help: This block creates a flat, single, square tile element. The square tile body is mass-less, so it will not have an effect on the dynamic simulation. This square tile element can be used as a graphic reference by itself, or as part of a composite graphic reference made of an array of interconnected tiles. The square tile is aligned with the XY plane, and the block provides frame connector ports to the middle points on each of the four sides of the body of the square - right (+X), left (-X), top (+Y) and bottom (-Y). All dimensions are in meters.
      settings: PortSchema="{\"entries\":[{\"content\":{\"sides\":[{\"content\":{\"connectorIds\":[\"LConn1\"]},\"type\":\"ConnectorPlacement.EquallySpacedRectSide\",\"uuid\":\"a971723f-ea37-4e9b-910b-501b94fb0ba2\"},{\"content\":{\"connectorIds\":[\"RConn1\"],\"side\":\"RIGHT\"},\"type\":\"ConnectorPlacement.EquallySpacedRectSide\",\"uuid\":\"e50175c1-005c-4b0b-bced-b882197eaab2\"},{\"content\":{\"connectorIds\":[\"LConn2\"],\"side\":\"TOP\"},\"type\":\"ConnectorPlacement.EquallySpacedRectSide\",\"uuid\":\"2a04a964-d53e-47ee-8c79-d53dd599bafe\"},{\"content\":{\"connectorIds\":[\"RConn2\"],\"side\":\"BOTTOM\"},\"type\":\"ConnectorPlacement.EquallySpacedRectSide\",\"uuid\":\"a0066dd6-a193-491c-afbe-bac00dfc3505\"}]},\"type\":\"ConnectorPlacement.EquallySpacedConnector\",\"uuid\":\"c80211c6-bb24-481b-97ca-2752015f3b18\"}],\"packageUris\":[\"http://schema.mathworks.com/mf0/Connector/19700101\"],\"version\":\"1.0\"}"
  Tile140 : Subsystem  mask(Square Tile){side=side, thickness=thick, color=color1, opacity=opacity}
      mask prompts: side "Side (m) :"; thickness "Thickness (m) :"; color "Color [RGB] :"; opacity "Opacity (0...1) :"
      mask help: This block creates a flat, single, square tile element. The square tile body is mass-less, so it will not have an effect on the dynamic simulation. This square tile element can be used as a graphic reference by itself, or as part of a composite graphic reference made of an array of interconnected tiles. The square tile is aligned with the XY plane, and the block provides frame connector ports to the middle points on each of the four sides of the body of the square - right (+X), left (-X), top (+Y) and bottom (-Y). All dimensions are in meters.
      settings: PortSchema="{\"entries\":[{\"content\":{\"sides\":[{\"content\":{\"connectorIds\":[\"LConn1\"]},\"type\":\"ConnectorPlacement.EquallySpacedRectSide\",\"uuid\":\"a971723f-ea37-4e9b-910b-501b94fb0ba2\"},{\"content\":{\"connectorIds\":[\"RConn1\"],\"side\":\"RIGHT\"},\"type\":\"ConnectorPlacement.EquallySpacedRectSide\",\"uuid\":\"e50175c1-005c-4b0b-bced-b882197eaab2\"},{\"content\":{\"connectorIds\":[\"LConn2\"],\"side\":\"TOP\"},\"type\":\"ConnectorPlacement.EquallySpacedRectSide\",\"uuid\":\"2a04a964-d53e-47ee-8c79-d53dd599bafe\"},{\"content\":{\"connectorIds\":[\"RConn2\"],\"side\":\"BOTTOM\"},\"type\":\"ConnectorPlacement.EquallySpacedRectSide\",\"uuid\":\"a0066dd6-a193-491c-afbe-bac00dfc3505\"}]},\"type\":\"ConnectorPlacement.EquallySpacedConnector\",\"uuid\":\"c80211c6-bb24-481b-97ca-2752015f3b18\"}],\"packageUris\":[\"http://schema.mathworks.com/mf0/Connector/19700101\"],\"version\":\"1.0\"}"
  Tile141 : Subsystem  mask(Square Tile){side=side, thickness=thick, color=color2, opacity=opacity}
      mask prompts: side "Side (m) :"; thickness "Thickness (m) :"; color "Color [RGB] :"; opacity "Opacity (0...1) :"
      mask help: This block creates a flat, single, square tile element. The square tile body is mass-less, so it will not have an effect on the dynamic simulation. This square tile element can be used as a graphic reference by itself, or as part of a composite graphic reference made of an array of interconnected tiles. The square tile is aligned with the XY plane, and the block provides frame connector ports to the middle points on each of the four sides of the body of the square - right (+X), left (-X), top (+Y) and bottom (-Y). All dimensions are in meters.
      settings: PortSchema="{\"entries\":[{\"content\":{\"sides\":[{\"content\":{\"connectorIds\":[\"LConn1\"]},\"type\":\"ConnectorPlacement.EquallySpacedRectSide\",\"uuid\":\"a971723f-ea37-4e9b-910b-501b94fb0ba2\"},{\"content\":{\"connectorIds\":[\"RConn1\"],\"side\":\"RIGHT\"},\"type\":\"ConnectorPlacement.EquallySpacedRectSide\",\"uuid\":\"e50175c1-005c-4b0b-bced-b882197eaab2\"},{\"content\":{\"connectorIds\":[\"LConn2\"],\"side\":\"TOP\"},\"type\":\"ConnectorPlacement.EquallySpacedRectSide\",\"uuid\":\"2a04a964-d53e-47ee-8c79-d53dd599bafe\"},{\"content\":{\"connectorIds\":[\"RConn2\"],\"side\":\"BOTTOM\"},\"type\":\"ConnectorPlacement.EquallySpacedRectSide\",\"uuid\":\"a0066dd6-a193-491c-afbe-bac00dfc3505\"}]},\"type\":\"ConnectorPlacement.EquallySpacedConnector\",\"uuid\":\"c80211c6-bb24-481b-97ca-2752015f3b18\"}],\"packageUris\":[\"http://schema.mathworks.com/mf0/Connector/19700101\"],\"version\":\"1.0\"}"
  Tile142 : Subsystem  mask(Square Tile){side=side, thickness=thick, color=color2, opacity=opacity}
      mask prompts: side "Side (m) :"; thickness "Thickness (m) :"; color "Color [RGB] :"; opacity "Opacity (0...1) :"
      mask help: This block creates a flat, single, square tile element. The square tile body is mass-less, so it will not have an effect on the dynamic simulation. This square tile element can be used as a graphic reference by itself, or as part of a composite graphic reference made of an array of interconnected tiles. The square tile is aligned with the XY plane, and the block provides frame connector ports to the middle points on each of the four sides of the body of the square - right (+X), left (-X), top (+Y) and bottom (-Y). All dimensions are in meters.
      settings: PortSchema="{\"entries\":[{\"content\":{\"sides\":[{\"content\":{\"connectorIds\":[\"LConn1\"]},\"type\":\"ConnectorPlacement.EquallySpacedRectSide\",\"uuid\":\"a971723f-ea37-4e9b-910b-501b94fb0ba2\"},{\"content\":{\"connectorIds\":[\"RConn1\"],\"side\":\"RIGHT\"},\"type\":\"ConnectorPlacement.EquallySpacedRectSide\",\"uuid\":\"e50175c1-005c-4b0b-bced-b882197eaab2\"},{\"content\":{\"connectorIds\":[\"LConn2\"],\"side\":\"TOP\"},\"type\":\"ConnectorPlacement.EquallySpacedRectSide\",\"uuid\":\"2a04a964-d53e-47ee-8c79-d53dd599bafe\"},{\"content\":{\"connectorIds\":[\"RConn2\"],\"side\":\"BOTTOM\"},\"type\":\"ConnectorPlacement.EquallySpacedRectSide\",\"uuid\":\"a0066dd6-a193-491c-afbe-bac00dfc3505\"}]},\"type\":\"ConnectorPlacement.EquallySpacedConnector\",\"uuid\":\"c80211c6-bb24-481b-97ca-2752015f3b18\"}],\"packageUris\":[\"http://schema.mathworks.com/mf0/Connector/19700101\"],\"version\":\"1.0\"}"
  Tile143 : Subsystem  mask(Square Tile){side=side, thickness=thick, color=color1, opacity=opacity}
      mask prompts: side "Side (m) :"; thickness "Thickness (m) :"; color "Color [RGB] :"; opacity "Opacity (0...1) :"
      mask help: This block creates a flat, single, square tile element. The square tile body is mass-less, so it will not have an effect on the dynamic simulation. This square tile element can be used as a graphic reference by itself, or as part of a composite graphic reference made of an array of interconnected tiles. The square tile is aligned with the XY plane, and the block provides frame connector ports to the middle points on each of the four sides of the body of the square - right (+X), left (-X), top (+Y) and bottom (-Y). All dimensions are in meters.
      settings: PortSchema="{\"entries\":[{\"content\":{\"sides\":[{\"content\":{\"connectorIds\":[\"LConn1\"]},\"type\":\"ConnectorPlacement.EquallySpacedRectSide\",\"uuid\":\"a971723f-ea37-4e9b-910b-501b94fb0ba2\"},{\"content\":{\"connectorIds\":[\"RConn1\"],\"side\":\"RIGHT\"},\"type\":\"ConnectorPlacement.EquallySpacedRectSide\",\"uuid\":\"e50175c1-005c-4b0b-bced-b882197eaab2\"},{\"content\":{\"connectorIds\":[\"LConn2\"],\"side\":\"TOP\"},\"type\":\"ConnectorPlacement.EquallySpacedRectSide\",\"uuid\":\"2a04a964-d53e-47ee-8c79-d53dd599bafe\"},{\"content\":{\"connectorIds\":[\"RConn2\"],\"side\":\"BOTTOM\"},\"type\":\"ConnectorPlacement.EquallySpacedRectSide\",\"uuid\":\"a0066dd6-a193-491c-afbe-bac00dfc3505\"}]},\"type\":\"ConnectorPlacement.EquallySpacedConnector\",\"uuid\":\"c80211c6-bb24-481b-97ca-2752015f3b18\"}],\"packageUris\":[\"http://schema.mathworks.com/mf0/Connector/19700101\"],\"version\":\"1.0\"}"
  Tile144 : Subsystem  mask(Square Tile){side=side, thickness=thick, color=color1, opacity=opacity}
      mask prompts: side "Side (m) :"; thickness "Thickness (m) :"; color "Color [RGB] :"; opacity "Opacity (0...1) :"
      mask help: This block creates a flat, single, square tile element. The square tile body is mass-less, so it will not have an effect on the dynamic simulation. This square tile element can be used as a graphic reference by itself, or as part of a composite graphic reference made of an array of interconnected tiles. The square tile is aligned with the XY plane, and the block provides frame connector ports to the middle points on each of the four sides of the body of the square - right (+X), left (-X), top (+Y) and bottom (-Y). All dimensions are in meters.
      settings: PortSchema="{\"entries\":[{\"content\":{\"sides\":[{\"content\":{\"connectorIds\":[\"LConn1\"]},\"type\":\"ConnectorPlacement.EquallySpacedRectSide\",\"uuid\":\"a971723f-ea37-4e9b-910b-501b94fb0ba2\"},{\"content\":{\"connectorIds\":[\"RConn1\"],\"side\":\"RIGHT\"},\"type\":\"ConnectorPlacement.EquallySpacedRectSide\",\"uuid\":\"e50175c1-005c-4b0b-bced-b882197eaab2\"},{\"content\":{\"connectorIds\":[\"LConn2\"],\"side\":\"TOP\"},\"type\":\"ConnectorPlacement.EquallySpacedRectSide\",\"uuid\":\"2a04a964-d53e-47ee-8c79-d53dd599bafe\"},{\"content\":{\"connectorIds\":[\"RConn2\"],\"side\":\"BOTTOM\"},\"type\":\"ConnectorPlacement.EquallySpacedRectSide\",\"uuid\":\"a0066dd6-a193-491c-afbe-bac00dfc3505\"}]},\"type\":\"ConnectorPlacement.EquallySpacedConnector\",\"uuid\":\"c80211c6-bb24-481b-97ca-2752015f3b18\"}],\"packageUris\":[\"http://schema.mathworks.com/mf0/Connector/19700101\"],\"version\":\"1.0\"}"
  Tile145 : Subsystem  mask(Square Tile){side=side, thickness=thick, color=color2, opacity=opacity}
      mask prompts: side "Side (m) :"; thickness "Thickness (m) :"; color "Color [RGB] :"; opacity "Opacity (0...1) :"
      mask help: This block creates a flat, single, square tile element. The square tile body is mass-less, so it will not have an effect on the dynamic simulation. This square tile element can be used as a graphic reference by itself, or as part of a composite graphic reference made of an array of interconnected tiles. The square tile is aligned with the XY plane, and the block provides frame connector ports to the middle points on each of the four sides of the body of the square - right (+X), left (-X), top (+Y) and bottom (-Y). All dimensions are in meters.
      settings: PortSchema="{\"entries\":[{\"content\":{\"sides\":[{\"content\":{\"connectorIds\":[\"LConn1\"]},\"type\":\"ConnectorPlacement.EquallySpacedRectSide\",\"uuid\":\"a971723f-ea37-4e9b-910b-501b94fb0ba2\"},{\"content\":{\"connectorIds\":[\"RConn1\"],\"side\":\"RIGHT\"},\"type\":\"ConnectorPlacement.EquallySpacedRectSide\",\"uuid\":\"e50175c1-005c-4b0b-bced-b882197eaab2\"},{\"content\":{\"connectorIds\":[\"LConn2\"],\"side\":\"TOP\"},\"type\":\"ConnectorPlacement.EquallySpacedRectSide\",\"uuid\":\"2a04a964-d53e-47ee-8c79-d53dd599bafe\"},{\"content\":{\"connectorIds\":[\"RConn2\"],\"side\":\"BOTTOM\"},\"type\":\"ConnectorPlacement.EquallySpacedRectSide\",\"uuid\":\"a0066dd6-a193-491c-afbe-bac00dfc3505\"}]},\"type\":\"ConnectorPlacement.EquallySpacedConnector\",\"uuid\":\"c80211c6-bb24-481b-97ca-2752015f3b18\"}],\"packageUris\":[\"http://schema.mathworks.com/mf0/Connector/19700101\"],\"version\":\"1.0\"}"
  Tile146 : Subsystem  mask(Square Tile){side=side, thickness=thick, color=color1, opacity=opacity}
      mask prompts: side "Side (m) :"; thickness "Thickness (m) :"; color "Color [RGB] :"; opacity "Opacity (0...1) :"
      mask help: This block creates a flat, single, square tile element. The square tile body is mass-less, so it will not have an effect on the dynamic simulation. This square tile element can be used as a graphic reference by itself, or as part of a composite graphic reference made of an array of interconnected tiles. The square tile is aligned with the XY plane, and the block provides frame connector ports to the middle points on each of the four sides of the body of the square - right (+X), left (-X), top (+Y) and bottom (-Y). All dimensions are in meters.
      settings: PortSchema="{\"entries\":[{\"content\":{\"sides\":[{\"content\":{\"connectorIds\":[\"LConn1\"]},\"type\":\"ConnectorPlacement.EquallySpacedRectSide\",\"uuid\":\"a971723f-ea37-4e9b-910b-501b94fb0ba2\"},{\"content\":{\"connectorIds\":[\"RConn1\"],\"side\":\"RIGHT\"},\"type\":\"ConnectorPlacement.EquallySpacedRectSide\",\"uuid\":\"e50175c1-005c-4b0b-bced-b882197eaab2\"},{\"content\":{\"connectorIds\":[\"LConn2\"],\"side\":\"TOP\"},\"type\":\"ConnectorPlacement.EquallySpacedRectSide\",\"uuid\":\"2a04a964-d53e-47ee-8c79-d53dd599bafe\"},{\"content\":{\"connectorIds\":[\"RConn2\"],\"side\":\"BOTTOM\"},\"type\":\"ConnectorPlacement.EquallySpacedRectSide\",\"uuid\":\"a0066dd6-a193-491c-afbe-bac00dfc3505\"}]},\"type\":\"ConnectorPlacement.EquallySpacedConnector\",\"uuid\":\"c80211c6-bb24-481b-97ca-2752015f3b18\"}],\"packageUris\":[\"http://schema.mathworks.com/mf0/Connector/19700101\"],\"version\":\"1.0\"}"
  Tile147 : Subsystem  mask(Square Tile){side=side, thickness=thick, color=color2, opacity=opacity}
      mask prompts: side "Side (m) :"; thickness "Thickness (m) :"; color "Color [RGB] :"; opacity "Opacity (0...1) :"
      mask help: This block creates a flat, single, square tile element. The square tile body is mass-less, so it will not have an effect on the dynamic simulation. This square tile element can be used as a graphic reference by itself, or as part of a composite graphic reference made of an array of interconnected tiles. The square tile is aligned with the XY plane, and the block provides frame connector ports to the middle points on each of the four sides of the body of the square - right (+X), left (-X), top (+Y) and bottom (-Y). All dimensions are in meters.
      settings: PortSchema="{\"entries\":[{\"content\":{\"sides\":[{\"content\":{\"connectorIds\":[\"LConn1\"]},\"type\":\"ConnectorPlacement.EquallySpacedRectSide\",\"uuid\":\"a971723f-ea37-4e9b-910b-501b94fb0ba2\"},{\"content\":{\"connectorIds\":[\"RConn1\"],\"side\":\"RIGHT\"},\"type\":\"ConnectorPlacement.EquallySpacedRectSide\",\"uuid\":\"e50175c1-005c-4b0b-bced-b882197eaab2\"},{\"content\":{\"connectorIds\":[\"LConn2\"],\"side\":\"TOP\"},\"type\":\"ConnectorPlacement.EquallySpacedRectSide\",\"uuid\":\"2a04a964-d53e-47ee-8c79-d53dd599bafe\"},{\"content\":{\"connectorIds\":[\"RConn2\"],\"side\":\"BOTTOM\"},\"type\":\"ConnectorPlacement.EquallySpacedRectSide\",\"uuid\":\"a0066dd6-a193-491c-afbe-bac00dfc3505\"}]},\"type\":\"ConnectorPlacement.EquallySpacedConnector\",\"uuid\":\"c80211c6-bb24-481b-97ca-2752015f3b18\"}],\"packageUris\":[\"http://schema.mathworks.com/mf0/Connector/19700101\"],\"version\":\"1.0\"}"
  Tile148 : Subsystem  mask(Square Tile){side=side, thickness=thick, color=color2, opacity=opacity}
      mask prompts: side "Side (m) :"; thickness "Thickness (m) :"; color "Color [RGB] :"; opacity "Opacity (0...1) :"
      mask help: This block creates a flat, single, square tile element. The square tile body is mass-less, so it will not have an effect on the dynamic simulation. This square tile element can be used as a graphic reference by itself, or as part of a composite graphic reference made of an array of interconnected tiles. The square tile is aligned with the XY plane, and the block provides frame connector ports to the middle points on each of the four sides of the body of the square - right (+X), left (-X), top (+Y) and bottom (-Y). All dimensions are in meters.
      settings: PortSchema="{\"entries\":[{\"content\":{\"sides\":[{\"content\":{\"connectorIds\":[\"LConn1\"]},\"type\":\"ConnectorPlacement.EquallySpacedRectSide\",\"uuid\":\"a971723f-ea37-4e9b-910b-501b94fb0ba2\"},{\"content\":{\"connectorIds\":[\"RConn1\"],\"side\":\"RIGHT\"},\"type\":\"ConnectorPlacement.EquallySpacedRectSide\",\"uuid\":\"e50175c1-005c-4b0b-bced-b882197eaab2\"},{\"content\":{\"connectorIds\":[\"LConn2\"],\"side\":\"TOP\"},\"type\":\"ConnectorPlacement.EquallySpacedRectSide\",\"uuid\":\"2a04a964-d53e-47ee-8c79-d53dd599bafe\"},{\"content\":{\"connectorIds\":[\"RConn2\"],\"side\":\"BOTTOM\"},\"type\":\"ConnectorPlacement.EquallySpacedRectSide\",\"uuid\":\"a0066dd6-a193-491c-afbe-bac00dfc3505\"}]},\"type\":\"ConnectorPlacement.EquallySpacedConnector\",\"uuid\":\"c80211c6-bb24-481b-97ca-2752015f3b18\"}],\"packageUris\":[\"http://schema.mathworks.com/mf0/Connector/19700101\"],\"version\":\"1.0\"}"
  Tile149 : Subsystem  mask(Square Tile){side=side, thickness=thick, color=color1, opacity=opacity}
      mask prompts: side "Side (m) :"; thickness "Thickness (m) :"; color "Color [RGB] :"; opacity "Opacity (0...1) :"
      mask help: This block creates a flat, single, square tile element. The square tile body is mass-less, so it will not have an effect on the dynamic simulation. This square tile element can be used as a graphic reference by itself, or as part of a composite graphic reference made of an array of interconnected tiles. The square tile is aligned with the XY plane, and the block provides frame connector ports to the middle points on each of the four sides of the body of the square - right (+X), left (-X), top (+Y) and bottom (-Y). All dimensions are in meters.
      settings: PortSchema="{\"entries\":[{\"content\":{\"sides\":[{\"content\":{\"connectorIds\":[\"LConn1\"]},\"type\":\"ConnectorPlacement.EquallySpacedRectSide\",\"uuid\":\"a971723f-ea37-4e9b-910b-501b94fb0ba2\"},{\"content\":{\"connectorIds\":[\"RConn1\"],\"side\":\"RIGHT\"},\"type\":\"ConnectorPlacement.EquallySpacedRectSide\",\"uuid\":\"e50175c1-005c-4b0b-bced-b882197eaab2\"},{\"content\":{\"connectorIds\":[\"LConn2\"],\"side\":\"TOP\"},\"type\":\"ConnectorPlacement.EquallySpacedRectSide\",\"uuid\":\"2a04a964-d53e-47ee-8c79-d53dd599bafe\"},{\"content\":{\"connectorIds\":[\"RConn2\"],\"side\":\"BOTTOM\"},\"type\":\"ConnectorPlacement.EquallySpacedRectSide\",\"uuid\":\"a0066dd6-a193-491c-afbe-bac00dfc3505\"}]},\"type\":\"ConnectorPlacement.EquallySpacedConnector\",\"uuid\":\"c80211c6-bb24-481b-97ca-2752015f3b18\"}],\"packageUris\":[\"http://schema.mathworks.com/mf0/Connector/19700101\"],\"version\":\"1.0\"}"
  Tile15 : Subsystem  mask(Square Tile){side=side, thickness=thick, color=color1, opacity=opacity}
      mask prompts: side "Side (m) :"; thickness "Thickness (m) :"; color "Color [RGB] :"; opacity "Opacity (0...1) :"
      mask help: This block creates a flat, single, square tile element. The square tile body is mass-less, so it will not have an effect on the dynamic simulation. This square tile element can be used as a graphic reference by itself, or as part of a composite graphic reference made of an array of interconnected tiles. The square tile is aligned with the XY plane, and the block provides frame connector ports to the middle points on each of the four sides of the body of the square - right (+X), left (-X), top (+Y) and bottom (-Y). All dimensions are in meters.
      settings: PortSchema="{\"entries\":[{\"content\":{\"sides\":[{\"content\":{\"connectorIds\":[\"LConn1\"]},\"type\":\"ConnectorPlacement.EquallySpacedRectSide\",\"uuid\":\"a971723f-ea37-4e9b-910b-501b94fb0ba2\"},{\"content\":{\"connectorIds\":[\"RConn1\"],\"side\":\"RIGHT\"},\"type\":\"ConnectorPlacement.EquallySpacedRectSide\",\"uuid\":\"e50175c1-005c-4b0b-bced-b882197eaab2\"},{\"content\":{\"connectorIds\":[\"LConn2\"],\"side\":\"TOP\"},\"type\":\"ConnectorPlacement.EquallySpacedRectSide\",\"uuid\":\"2a04a964-d53e-47ee-8c79-d53dd599bafe\"},{\"content\":{\"connectorIds\":[\"RConn2\"],\"side\":\"BOTTOM\"},\"type\":\"ConnectorPlacement.EquallySpacedRectSide\",\"uuid\":\"a0066dd6-a193-491c-afbe-bac00dfc3505\"}]},\"type\":\"ConnectorPlacement.EquallySpacedConnector\",\"uuid\":\"c80211c6-bb24-481b-97ca-2752015f3b18\"}],\"packageUris\":[\"http://schema.mathworks.com/mf0/Connector/19700101\"],\"version\":\"1.0\"}"
  Tile150 : Subsystem  mask(Square Tile){side=side, thickness=thick, color=color2, opacity=opacity}
      mask prompts: side "Side (m) :"; thickness "Thickness (m) :"; color "Color [RGB] :"; opacity "Opacity (0...1) :"
      mask help: This block creates a flat, single, square tile element. The square tile body is mass-less, so it will not have an effect on the dynamic simulation. This square tile element can be used as a graphic reference by itself, or as part of a composite graphic reference made of an array of interconnected tiles. The square tile is aligned with the XY plane, and the block provides frame connector ports to the middle points on each of the four sides of the body of the square - right (+X), left (-X), top (+Y) and bottom (-Y). All dimensions are in meters.
      settings: PortSchema="{\"entries\":[{\"content\":{\"sides\":[{\"content\":{\"connectorIds\":[\"LConn1\"]},\"type\":\"ConnectorPlacement.EquallySpacedRectSide\",\"uuid\":\"a971723f-ea37-4e9b-910b-501b94fb0ba2\"},{\"content\":{\"connectorIds\":[\"RConn1\"],\"side\":\"RIGHT\"},\"type\":\"ConnectorPlacement.EquallySpacedRectSide\",\"uuid\":\"e50175c1-005c-4b0b-bced-b882197eaab2\"},{\"content\":{\"connectorIds\":[\"LConn2\"],\"side\":\"TOP\"},\"type\":\"ConnectorPlacement.EquallySpacedRectSide\",\"uuid\":\"2a04a964-d53e-47ee-8c79-d53dd599bafe\"},{\"content\":{\"connectorIds\":[\"RConn2\"],\"side\":\"BOTTOM\"},\"type\":\"ConnectorPlacement.EquallySpacedRectSide\",\"uuid\":\"a0066dd6-a193-491c-afbe-bac00dfc3505\"}]},\"type\":\"ConnectorPlacement.EquallySpacedConnector\",\"uuid\":\"c80211c6-bb24-481b-97ca-2752015f3b18\"}],\"packageUris\":[\"http://schema.mathworks.com/mf0/Connector/19700101\"],\"version\":\"1.0\"}"
  Tile151 : Subsystem  mask(Square Tile){side=side, thickness=thick, color=color1, opacity=opacity}
      mask prompts: side "Side (m) :"; thickness "Thickness (m) :"; color "Color [RGB] :"; opacity "Opacity (0...1) :"
      mask help: This block creates a flat, single, square tile element. The square tile body is mass-less, so it will not have an effect on the dynamic simulation. This square tile element can be used as a graphic reference by itself, or as part of a composite graphic reference made of an array of interconnected tiles. The square tile is aligned with the XY plane, and the block provides frame connector ports to the middle points on each of the four sides of the body of the square - right (+X), left (-X), top (+Y) and bottom (-Y). All dimensions are in meters.
      settings: PortSchema="{\"entries\":[{\"content\":{\"sides\":[{\"content\":{\"connectorIds\":[\"LConn1\"]},\"type\":\"ConnectorPlacement.EquallySpacedRectSide\",\"uuid\":\"a971723f-ea37-4e9b-910b-501b94fb0ba2\"},{\"content\":{\"connectorIds\":[\"RConn1\"],\"side\":\"RIGHT\"},\"type\":\"ConnectorPlacement.EquallySpacedRectSide\",\"uuid\":\"e50175c1-005c-4b0b-bced-b882197eaab2\"},{\"content\":{\"connectorIds\":[\"LConn2\"],\"side\":\"TOP\"},\"type\":\"ConnectorPlacement.EquallySpacedRectSide\",\"uuid\":\"2a04a964-d53e-47ee-8c79-d53dd599bafe\"},{\"content\":{\"connectorIds\":[\"RConn2\"],\"side\":\"BOTTOM\"},\"type\":\"ConnectorPlacement.EquallySpacedRectSide\",\"uuid\":\"a0066dd6-a193-491c-afbe-bac00dfc3505\"}]},\"type\":\"ConnectorPlacement.EquallySpacedConnector\",\"uuid\":\"c80211c6-bb24-481b-97ca-2752015f3b18\"}],\"packageUris\":[\"http://schema.mathworks.com/mf0/Connector/19700101\"],\"version\":\"1.0\"}"
  Tile152 : Subsystem  mask(Square Tile){side=side, thickness=thick, color=color1, opacity=opacity}
      mask prompts: side "Side (m) :"; thickness "Thickness (m) :"; color "Color [RGB] :"; opacity "Opacity (0...1) :"
      mask help: This block creates a flat, single, square tile element. The square tile body is mass-less, so it will not have an effect on the dynamic simulation. This square tile element can be used as a graphic reference by itself, or as part of a composite graphic reference made of an array of interconnected tiles. The square tile is aligned with the XY plane, and the block provides frame connector ports to the middle points on each of the four sides of the body of the square - right (+X), left (-X), top (+Y) and bottom (-Y). All dimensions are in meters.
      settings: PortSchema="{\"entries\":[{\"content\":{\"sides\":[{\"content\":{\"connectorIds\":[\"LConn1\"]},\"type\":\"ConnectorPlacement.EquallySpacedRectSide\",\"uuid\":\"a971723f-ea37-4e9b-910b-501b94fb0ba2\"},{\"content\":{\"connectorIds\":[\"RConn1\"],\"side\":\"RIGHT\"},\"type\":\"ConnectorPlacement.EquallySpacedRectSide\",\"uuid\":\"e50175c1-005c-4b0b-bced-b882197eaab2\"},{\"content\":{\"connectorIds\":[\"LConn2\"],\"side\":\"TOP\"},\"type\":\"ConnectorPlacement.EquallySpacedRectSide\",\"uuid\":\"2a04a964-d53e-47ee-8c79-d53dd599bafe\"},{\"content\":{\"connectorIds\":[\"RConn2\"],\"side\":\"BOTTOM\"},\"type\":\"ConnectorPlacement.EquallySpacedRectSide\",\"uuid\":\"a0066dd6-a193-491c-afbe-bac00dfc3505\"}]},\"type\":\"ConnectorPlacement.EquallySpacedConnector\",\"uuid\":\"c80211c6-bb24-481b-97ca-2752015f3b18\"}],\"packageUris\":[\"http://schema.mathworks.com/mf0/Connector/19700101\"],\"version\":\"1.0\"}"
  Tile153 : Subsystem  mask(Square Tile){side=side, thickness=thick, color=color2, opacity=opacity}
      mask prompts: side "Side (m) :"; thickness "Thickness (m) :"; color "Color [RGB] :"; opacity "Opacity (0...1) :"
      mask help: This block creates a flat, single, square tile element. The square tile body is mass-less, so it will not have an effect on the dynamic simulation. This square tile element can be used as a graphic reference by itself, or as part of a composite graphic reference made of an array of interconnected tiles. The square tile is aligned with the XY plane, and the block provides frame connector ports to the middle points on each of the four sides of the body of the square - right (+X), left (-X), top (+Y) and bottom (-Y). All dimensions are in meters.
      settings: PortSchema="{\"entries\":[{\"content\":{\"sides\":[{\"content\":{\"connectorIds\":[\"LConn1\"]},\"type\":\"ConnectorPlacement.EquallySpacedRectSide\",\"uuid\":\"a971723f-ea37-4e9b-910b-501b94fb0ba2\"},{\"content\":{\"connectorIds\":[\"RConn1\"],\"side\":\"RIGHT\"},\"type\":\"ConnectorPlacement.EquallySpacedRectSide\",\"uuid\":\"e50175c1-005c-4b0b-bced-b882197eaab2\"},{\"content\":{\"connectorIds\":[\"LConn2\"],\"side\":\"TOP\"},\"type\":\"ConnectorPlacement.EquallySpacedRectSide\",\"uuid\":\"2a04a964-d53e-47ee-8c79-d53dd599bafe\"},{\"content\":{\"connectorIds\":[\"RConn2\"],\"side\":\"BOTTOM\"},\"type\":\"ConnectorPlacement.EquallySpacedRectSide\",\"uuid\":\"a0066dd6-a193-491c-afbe-bac00dfc3505\"}]},\"type\":\"ConnectorPlacement.EquallySpacedConnector\",\"uuid\":\"c80211c6-bb24-481b-97ca-2752015f3b18\"}],\"packageUris\":[\"http://schema.mathworks.com/mf0/Connector/19700101\"],\"version\":\"1.0\"}"
  Tile154 : Subsystem  mask(Square Tile){side=side, thickness=thick, color=color1, opacity=opacity}
      mask prompts: side "Side (m) :"; thickness "Thickness (m) :"; color "Color [RGB] :"; opacity "Opacity (0...1) :"
      mask help: This block creates a flat, single, square tile element. The square tile body is mass-less, so it will not have an effect on the dynamic simulation. This square tile element can be used as a graphic reference by itself, or as part of a composite graphic reference made of an array of interconnected tiles. The square tile is aligned with the XY plane, and the block provides frame connector ports to the middle points on each of the four sides of the body of the square - right (+X), left (-X), top (+Y) and bottom (-Y). All dimensions are in meters.
      settings: PortSchema="{\"entries\":[{\"content\":{\"sides\":[{\"content\":{\"connectorIds\":[\"LConn1\"]},\"type\":\"ConnectorPlacement.EquallySpacedRectSide\",\"uuid\":\"a971723f-ea37-4e9b-910b-501b94fb0ba2\"},{\"content\":{\"connectorIds\":[\"RConn1\"],\"side\":\"RIGHT\"},\"type\":\"ConnectorPlacement.EquallySpacedRectSide\",\"uuid\":\"e50175c1-005c-4b0b-bced-b882197eaab2\"},{\"content\":{\"connectorIds\":[\"LConn2\"],\"side\":\"TOP\"},\"type\":\"ConnectorPlacement.EquallySpacedRectSide\",\"uuid\":\"2a04a964-d53e-47ee-8c79-d53dd599bafe\"},{\"content\":{\"connectorIds\":[\"RConn2\"],\"side\":\"BOTTOM\"},\"type\":\"ConnectorPlacement.EquallySpacedRectSide\",\"uuid\":\"a0066dd6-a193-491c-afbe-bac00dfc3505\"}]},\"type\":\"ConnectorPlacement.EquallySpacedConnector\",\"uuid\":\"c80211c6-bb24-481b-97ca-2752015f3b18\"}],\"packageUris\":[\"http://schema.mathworks.com/mf0/Connector/19700101\"],\"version\":\"1.0\"}"
  Tile155 : Subsystem  mask(Square Tile){side=side, thickness=thick, color=color1, opacity=opacity}
      mask prompts: side "Side (m) :"; thickness "Thickness (m) :"; color "Color [RGB] :"; opacity "Opacity (0...1) :"
      mask help: This block creates a flat, single, square tile element. The square tile body is mass-less, so it will not have an effect on the dynamic simulation. This square tile element can be used as a graphic reference by itself, or as part of a composite graphic reference made of an array of interconnected tiles. The square tile is aligned with the XY plane, and the block provides frame connector ports to the middle points on each of the four sides of the body of the square - right (+X), left (-X), top (+Y) and bottom (-Y). All dimensions are in meters.
      settings: PortSchema="{\"entries\":[{\"content\":{\"sides\":[{\"content\":{\"connectorIds\":[\"LConn1\"]},\"type\":\"ConnectorPlacement.EquallySpacedRectSide\",\"uuid\":\"a971723f-ea37-4e9b-910b-501b94fb0ba2\"},{\"content\":{\"connectorIds\":[\"RConn1\"],\"side\":\"RIGHT\"},\"type\":\"ConnectorPlacement.EquallySpacedRectSide\",\"uuid\":\"e50175c1-005c-4b0b-bced-b882197eaab2\"},{\"content\":{\"connectorIds\":[\"LConn2\"],\"side\":\"TOP\"},\"type\":\"ConnectorPlacement.EquallySpacedRectSide\",\"uuid\":\"2a04a964-d53e-47ee-8c79-d53dd599bafe\"},{\"content\":{\"connectorIds\":[\"RConn2\"],\"side\":\"BOTTOM\"},\"type\":\"ConnectorPlacement.EquallySpacedRectSide\",\"uuid\":\"a0066dd6-a193-491c-afbe-bac00dfc3505\"}]},\"type\":\"ConnectorPlacement.EquallySpacedConnector\",\"uuid\":\"c80211c6-bb24-481b-97ca-2752015f3b18\"}],\"packageUris\":[\"http://schema.mathworks.com/mf0/Connector/19700101\"],\"version\":\"1.0\"}"
  Tile156 : Subsystem  mask(Square Tile){side=side, thickness=thick, color=color2, opacity=opacity}
      mask prompts: side "Side (m) :"; thickness "Thickness (m) :"; color "Color [RGB] :"; opacity "Opacity (0...1) :"
      mask help: This block creates a flat, single, square tile element. The square tile body is mass-less, so it will not have an effect on the dynamic simulation. This square tile element can be used as a graphic reference by itself, or as part of a composite graphic reference made of an array of interconnected tiles. The square tile is aligned with the XY plane, and the block provides frame connector ports to the middle points on each of the four sides of the body of the square - right (+X), left (-X), top (+Y) and bottom (-Y). All dimensions are in meters.
      settings: PortSchema="{\"entries\":[{\"content\":{\"sides\":[{\"content\":{\"connectorIds\":[\"LConn1\"]},\"type\":\"ConnectorPlacement.EquallySpacedRectSide\",\"uuid\":\"a971723f-ea37-4e9b-910b-501b94fb0ba2\"},{\"content\":{\"connectorIds\":[\"RConn1\"],\"side\":\"RIGHT\"},\"type\":\"ConnectorPlacement.EquallySpacedRectSide\",\"uuid\":\"e50175c1-005c-4b0b-bced-b882197eaab2\"},{\"content\":{\"connectorIds\":[\"LConn2\"],\"side\":\"TOP\"},\"type\":\"ConnectorPlacement.EquallySpacedRectSide\",\"uuid\":\"2a04a964-d53e-47ee-8c79-d53dd599bafe\"},{\"content\":{\"connectorIds\":[\"RConn2\"],\"side\":\"BOTTOM\"},\"type\":\"ConnectorPlacement.EquallySpacedRectSide\",\"uuid\":\"a0066dd6-a193-491c-afbe-bac00dfc3505\"}]},\"type\":\"ConnectorPlacement.EquallySpacedConnector\",\"uuid\":\"c80211c6-bb24-481b-97ca-2752015f3b18\"}],\"packageUris\":[\"http://schema.mathworks.com/mf0/Connector/19700101\"],\"version\":\"1.0\"}"
  Tile157 : Subsystem  mask(Square Tile){side=side, thickness=thick, color=color2, opacity=opacity}
      mask prompts: side "Side (m) :"; thickness "Thickness (m) :"; color "Color [RGB] :"; opacity "Opacity (0...1) :"
      mask help: This block creates a flat, single, square tile element. The square tile body is mass-less, so it will not have an effect on the dynamic simulation. This square tile element can be used as a graphic reference by itself, or as part of a composite graphic reference made of an array of interconnected tiles. The square tile is aligned with the XY plane, and the block provides frame connector ports to the middle points on each of the four sides of the body of the square - right (+X), left (-X), top (+Y) and bottom (-Y). All dimensions are in meters.
      settings: PortSchema="{\"entries\":[{\"content\":{\"sides\":[{\"content\":{\"connectorIds\":[\"LConn1\"]},\"type\":\"ConnectorPlacement.EquallySpacedRectSide\",\"uuid\":\"a971723f-ea37-4e9b-910b-501b94fb0ba2\"},{\"content\":{\"connectorIds\":[\"RConn1\"],\"side\":\"RIGHT\"},\"type\":\"ConnectorPlacement.EquallySpacedRectSide\",\"uuid\":\"e50175c1-005c-4b0b-bced-b882197eaab2\"},{\"content\":{\"connectorIds\":[\"LConn2\"],\"side\":\"TOP\"},\"type\":\"ConnectorPlacement.EquallySpacedRectSide\",\"uuid\":\"2a04a964-d53e-47ee-8c79-d53dd599bafe\"},{\"content\":{\"connectorIds\":[\"RConn2\"],\"side\":\"BOTTOM\"},\"type\":\"ConnectorPlacement.EquallySpacedRectSide\",\"uuid\":\"a0066dd6-a193-491c-afbe-bac00dfc3505\"}]},\"type\":\"ConnectorPlacement.EquallySpacedConnector\",\"uuid\":\"c80211c6-bb24-481b-97ca-2752015f3b18\"}],\"packageUris\":[\"http://schema.mathworks.com/mf0/Connector/19700101\"],\"version\":\"1.0\"}"
  Tile158 : Subsystem  mask(Square Tile){side=side, thickness=thick, color=color2, opacity=opacity}
      mask prompts: side "Side (m) :"; thickness "Thickness (m) :"; color "Color [RGB] :"; opacity "Opacity (0...1) :"
      mask help: This block creates a flat, single, square tile element. The square tile body is mass-less, so it will not have an effect on the dynamic simulation. This square tile element can be used as a graphic reference by itself, or as part of a composite graphic reference made of an array of interconnected tiles. The square tile is aligned with the XY plane, and the block provides frame connector ports to the middle points on each of the four sides of the body of the square - right (+X), left (-X), top (+Y) and bottom (-Y). All dimensions are in meters.
      settings: PortSchema="{\"entries\":[{\"content\":{\"sides\":[{\"content\":{\"connectorIds\":[\"LConn1\"]},\"type\":\"ConnectorPlacement.EquallySpacedRectSide\",\"uuid\":\"a971723f-ea37-4e9b-910b-501b94fb0ba2\"},{\"content\":{\"connectorIds\":[\"RConn1\"],\"side\":\"RIGHT\"},\"type\":\"ConnectorPlacement.EquallySpacedRectSide\",\"uuid\":\"e50175c1-005c-4b0b-bced-b882197eaab2\"},{\"content\":{\"connectorIds\":[\"LConn2\"],\"side\":\"TOP\"},\"type\":\"ConnectorPlacement.EquallySpacedRectSide\",\"uuid\":\"2a04a964-d53e-47ee-8c79-d53dd599bafe\"},{\"content\":{\"connectorIds\":[\"RConn2\"],\"side\":\"BOTTOM\"},\"type\":\"ConnectorPlacement.EquallySpacedRectSide\",\"uuid\":\"a0066dd6-a193-491c-afbe-bac00dfc3505\"}]},\"type\":\"ConnectorPlacement.EquallySpacedConnector\",\"uuid\":\"c80211c6-bb24-481b-97ca-2752015f3b18\"}],\"packageUris\":[\"http://schema.mathworks.com/mf0/Connector/19700101\"],\"version\":\"1.0\"}"
  Tile159 : Subsystem  mask(Square Tile){side=side, thickness=thick, color=color1, opacity=opacity}
      mask prompts: side "Side (m) :"; thickness "Thickness (m) :"; color "Color [RGB] :"; opacity "Opacity (0...1) :"
      mask help: This block creates a flat, single, square tile element. The square tile body is mass-less, so it will not have an effect on the dynamic simulation. This square tile element can be used as a graphic reference by itself, or as part of a composite graphic reference made of an array of interconnected tiles. The square tile is aligned with the XY plane, and the block provides frame connector ports to the middle points on each of the four sides of the body of the square - right (+X), left (-X), top (+Y) and bottom (-Y). All dimensions are in meters.
      settings: PortSchema="{\"entries\":[{\"content\":{\"sides\":[{\"content\":{\"connectorIds\":[\"LConn1\"]},\"type\":\"ConnectorPlacement.EquallySpacedRectSide\",\"uuid\":\"a971723f-ea37-4e9b-910b-501b94fb0ba2\"},{\"content\":{\"connectorIds\":[\"RConn1\"],\"side\":\"RIGHT\"},\"type\":\"ConnectorPlacement.EquallySpacedRectSide\",\"uuid\":\"e50175c1-005c-4b0b-bced-b882197eaab2\"},{\"content\":{\"connectorIds\":[\"LConn2\"],\"side\":\"TOP\"},\"type\":\"ConnectorPlacement.EquallySpacedRectSide\",\"uuid\":\"2a04a964-d53e-47ee-8c79-d53dd599bafe\"},{\"content\":{\"connectorIds\":[\"RConn2\"],\"side\":\"BOTTOM\"},\"type\":\"ConnectorPlacement.EquallySpacedRectSide\",\"uuid\":\"a0066dd6-a193-491c-afbe-bac00dfc3505\"}]},\"type\":\"ConnectorPlacement.EquallySpacedConnector\",\"uuid\":\"c80211c6-bb24-481b-97ca-2752015f3b18\"}],\"packageUris\":[\"http://schema.mathworks.com/mf0/Connector/19700101\"],\"version\":\"1.0\"}"
  Tile16 : Subsystem  mask(Square Tile){side=side, thickness=thick, color=color2, opacity=opacity}
      mask prompts: side "Side (m) :"; thickness "Thickness (m) :"; color "Color [RGB] :"; opacity "Opacity (0...1) :"
      mask help: This block creates a flat, single, square tile element. The square tile body is mass-less, so it will not have an effect on the dynamic simulation. This square tile element can be used as a graphic reference by itself, or as part of a composite graphic reference made of an array of interconnected tiles. The square tile is aligned with the XY plane, and the block provides frame connector ports to the middle points on each of the four sides of the body of the square - right (+X), left (-X), top (+Y) and bottom (-Y). All dimensions are in meters.
      settings: PortSchema="{\"entries\":[{\"content\":{\"sides\":[{\"content\":{\"connectorIds\":[\"LConn1\"]},\"type\":\"ConnectorPlacement.EquallySpacedRectSide\",\"uuid\":\"a971723f-ea37-4e9b-910b-501b94fb0ba2\"},{\"content\":{\"connectorIds\":[\"RConn1\"],\"side\":\"RIGHT\"},\"type\":\"ConnectorPlacement.EquallySpacedRectSide\",\"uuid\":\"e50175c1-005c-4b0b-bced-b882197eaab2\"},{\"content\":{\"connectorIds\":[\"LConn2\"],\"side\":\"TOP\"},\"type\":\"ConnectorPlacement.EquallySpacedRectSide\",\"uuid\":\"2a04a964-d53e-47ee-8c79-d53dd599bafe\"},{\"content\":{\"connectorIds\":[\"RConn2\"],\"side\":\"BOTTOM\"},\"type\":\"ConnectorPlacement.EquallySpacedRectSide\",\"uuid\":\"a0066dd6-a193-491c-afbe-bac00dfc3505\"}]},\"type\":\"ConnectorPlacement.EquallySpacedConnector\",\"uuid\":\"c80211c6-bb24-481b-97ca-2752015f3b18\"}],\"packageUris\":[\"http://schema.mathworks.com/mf0/Connector/19700101\"],\"version\":\"1.0\"}"
  Tile160 : Subsystem  mask(Square Tile){side=side, thickness=thick, color=color1, opacity=opacity}
      mask prompts: side "Side (m) :"; thickness "Thickness (m) :"; color "Color [RGB] :"; opacity "Opacity (0...1) :"
      mask help: This block creates a flat, single, square tile element. The square tile body is mass-less, so it will not have an effect on the dynamic simulation. This square tile element can be used as a graphic reference by itself, or as part of a composite graphic reference made of an array of interconnected tiles. The square tile is aligned with the XY plane, and the block provides frame connector ports to the middle points on each of the four sides of the body of the square - right (+X), left (-X), top (+Y) and bottom (-Y). All dimensions are in meters.
      settings: PortSchema="{\"entries\":[{\"content\":{\"sides\":[{\"content\":{\"connectorIds\":[\"LConn1\"]},\"type\":\"ConnectorPlacement.EquallySpacedRectSide\",\"uuid\":\"a971723f-ea37-4e9b-910b-501b94fb0ba2\"},{\"content\":{\"connectorIds\":[\"RConn1\"],\"side\":\"RIGHT\"},\"type\":\"ConnectorPlacement.EquallySpacedRectSide\",\"uuid\":\"e50175c1-005c-4b0b-bced-b882197eaab2\"},{\"content\":{\"connectorIds\":[\"LConn2\"],\"side\":\"TOP\"},\"type\":\"ConnectorPlacement.EquallySpacedRectSide\",\"uuid\":\"2a04a964-d53e-47ee-8c79-d53dd599bafe\"},{\"content\":{\"connectorIds\":[\"RConn2\"],\"side\":\"BOTTOM\"},\"type\":\"ConnectorPlacement.EquallySpacedRectSide\",\"uuid\":\"a0066dd6-a193-491c-afbe-bac00dfc3505\"}]},\"type\":\"ConnectorPlacement.EquallySpacedConnector\",\"uuid\":\"c80211c6-bb24-481b-97ca-2752015f3b18\"}],\"packageUris\":[\"http://schema.mathworks.com/mf0/Connector/19700101\"],\"version\":\"1.0\"}"
  Tile161 : Subsystem  mask(Square Tile){side=side, thickness=thick, color=color2, opacity=opacity}
      mask prompts: side "Side (m) :"; thickness "Thickness (m) :"; color "Color [RGB] :"; opacity "Opacity (0...1) :"
      mask help: This block creates a flat, single, square tile element. The square tile body is mass-less, so it will not have an effect on the dynamic simulation. This square tile element can be used as a graphic reference by itself, or as part of a composite graphic reference made of an array of interconnected tiles. The square tile is aligned with the XY plane, and the block provides frame connector ports to the middle points on each of the four sides of the body of the square - right (+X), left (-X), top (+Y) and bottom (-Y). All dimensions are in meters.
      settings: PortSchema="{\"entries\":[{\"content\":{\"sides\":[{\"content\":{\"connectorIds\":[\"LConn1\"]},\"type\":\"ConnectorPlacement.EquallySpacedRectSide\",\"uuid\":\"a971723f-ea37-4e9b-910b-501b94fb0ba2\"},{\"content\":{\"connectorIds\":[\"RConn1\"],\"side\":\"RIGHT\"},\"type\":\"ConnectorPlacement.EquallySpacedRectSide\",\"uuid\":\"e50175c1-005c-4b0b-bced-b882197eaab2\"},{\"content\":{\"connectorIds\":[\"LConn2\"],\"side\":\"TOP\"},\"type\":\"ConnectorPlacement.EquallySpacedRectSide\",\"uuid\":\"2a04a964-d53e-47ee-8c79-d53dd599bafe\"},{\"content\":{\"connectorIds\":[\"RConn2\"],\"side\":\"BOTTOM\"},\"type\":\"ConnectorPlacement.EquallySpacedRectSide\",\"uuid\":\"a0066dd6-a193-491c-afbe-bac00dfc3505\"}]},\"type\":\"ConnectorPlacement.EquallySpacedConnector\",\"uuid\":\"c80211c6-bb24-481b-97ca-2752015f3b18\"}],\"packageUris\":[\"http://schema.mathworks.com/mf0/Connector/19700101\"],\"version\":\"1.0\"}"
  Tile162 : Subsystem  mask(Square Tile){side=side, thickness=thick, color=color1, opacity=opacity}
      mask prompts: side "Side (m) :"; thickness "Thickness (m) :"; color "Color [RGB] :"; opacity "Opacity (0...1) :"
      mask help: This block creates a flat, single, square tile element. The square tile body is mass-less, so it will not have an effect on the dynamic simulation. This square tile element can be used as a graphic reference by itself, or as part of a composite graphic reference made of an array of interconnected tiles. The square tile is aligned with the XY plane, and the block provides frame connector ports to the middle points on each of the four sides of the body of the square - right (+X), left (-X), top (+Y) and bottom (-Y). All dimensions are in meters.
      settings: PortSchema="{\"entries\":[{\"content\":{\"sides\":[{\"content\":{\"connectorIds\":[\"LConn1\"]},\"type\":\"ConnectorPlacement.EquallySpacedRectSide\",\"uuid\":\"a971723f-ea37-4e9b-910b-501b94fb0ba2\"},{\"content\":{\"connectorIds\":[\"RConn1\"],\"side\":\"RIGHT\"},\"type\":\"ConnectorPlacement.EquallySpacedRectSide\",\"uuid\":\"e50175c1-005c-4b0b-bced-b882197eaab2\"},{\"content\":{\"connectorIds\":[\"LConn2\"],\"side\":\"TOP\"},\"type\":\"ConnectorPlacement.EquallySpacedRectSide\",\"uuid\":\"2a04a964-d53e-47ee-8c79-d53dd599bafe\"},{\"content\":{\"connectorIds\":[\"RConn2\"],\"side\":\"BOTTOM\"},\"type\":\"ConnectorPlacement.EquallySpacedRectSide\",\"uuid\":\"a0066dd6-a193-491c-afbe-bac00dfc3505\"}]},\"type\":\"ConnectorPlacement.EquallySpacedConnector\",\"uuid\":\"c80211c6-bb24-481b-97ca-2752015f3b18\"}],\"packageUris\":[\"http://schema.mathworks.com/mf0/Connector/19700101\"],\"version\":\"1.0\"}"
  Tile163 : Subsystem  mask(Square Tile){side=side, thickness=thick, color=color1, opacity=opacity}
      mask prompts: side "Side (m) :"; thickness "Thickness (m) :"; color "Color [RGB] :"; opacity "Opacity (0...1) :"
      mask help: This block creates a flat, single, square tile element. The square tile body is mass-less, so it will not have an effect on the dynamic simulation. This square tile element can be used as a graphic reference by itself, or as part of a composite graphic reference made of an array of interconnected tiles. The square tile is aligned with the XY plane, and the block provides frame connector ports to the middle points on each of the four sides of the body of the square - right (+X), left (-X), top (+Y) and bottom (-Y). All dimensions are in meters.
      settings: PortSchema="{\"entries\":[{\"content\":{\"sides\":[{\"content\":{\"connectorIds\":[\"LConn1\"]},\"type\":\"ConnectorPlacement.EquallySpacedRectSide\",\"uuid\":\"a971723f-ea37-4e9b-910b-501b94fb0ba2\"},{\"content\":{\"connectorIds\":[\"RConn1\"],\"side\":\"RIGHT\"},\"type\":\"ConnectorPlacement.EquallySpacedRectSide\",\"uuid\":\"e50175c1-005c-4b0b-bced-b882197eaab2\"},{\"content\":{\"connectorIds\":[\"LConn2\"],\"side\":\"TOP\"},\"type\":\"ConnectorPlacement.EquallySpacedRectSide\",\"uuid\":\"2a04a964-d53e-47ee-8c79-d53dd599bafe\"},{\"content\":{\"connectorIds\":[\"RConn2\"],\"side\":\"BOTTOM\"},\"type\":\"ConnectorPlacement.EquallySpacedRectSide\",\"uuid\":\"a0066dd6-a193-491c-afbe-bac00dfc3505\"}]},\"type\":\"ConnectorPlacement.EquallySpacedConnector\",\"uuid\":\"c80211c6-bb24-481b-97ca-2752015f3b18\"}],\"packageUris\":[\"http://schema.mathworks.com/mf0/Connector/19700101\"],\"version\":\"1.0\"}"
  Tile164 : Subsystem  mask(Square Tile){side=side, thickness=thick, color=color2, opacity=opacity}
      mask prompts: side "Side (m) :"; thickness "Thickness (m) :"; color "Color [RGB] :"; opacity "Opacity (0...1) :"
      mask help: This block creates a flat, single, square tile element. The square tile body is mass-less, so it will not have an effect on the dynamic simulation. This square tile element can be used as a graphic reference by itself, or as part of a composite graphic reference made of an array of interconnected tiles. The square tile is aligned with the XY plane, and the block provides frame connector ports to the middle points on each of the four sides of the body of the square - right (+X), left (-X), top (+Y) and bottom (-Y). All dimensions are in meters.
      settings: PortSchema="{\"entries\":[{\"content\":{\"sides\":[{\"content\":{\"connectorIds\":[\"LConn1\"]},\"type\":\"ConnectorPlacement.EquallySpacedRectSide\",\"uuid\":\"a971723f-ea37-4e9b-910b-501b94fb0ba2\"},{\"content\":{\"connectorIds\":[\"RConn1\"],\"side\":\"RIGHT\"},\"type\":\"ConnectorPlacement.EquallySpacedRectSide\",\"uuid\":\"e50175c1-005c-4b0b-bced-b882197eaab2\"},{\"content\":{\"connectorIds\":[\"LConn2\"],\"side\":\"TOP\"},\"type\":\"ConnectorPlacement.EquallySpacedRectSide\",\"uuid\":\"2a04a964-d53e-47ee-8c79-d53dd599bafe\"},{\"content\":{\"connectorIds\":[\"RConn2\"],\"side\":\"BOTTOM\"},\"type\":\"ConnectorPlacement.EquallySpacedRectSide\",\"uuid\":\"a0066dd6-a193-491c-afbe-bac00dfc3505\"}]},\"type\":\"ConnectorPlacement.EquallySpacedConnector\",\"uuid\":\"c80211c6-bb24-481b-97ca-2752015f3b18\"}],\"packageUris\":[\"http://schema.mathworks.com/mf0/Connector/19700101\"],\"version\":\"1.0\"}"
  Tile165 : Subsystem  mask(Square Tile){side=side, thickness=thick, color=color2, opacity=opacity}
      mask prompts: side "Side (m) :"; thickness "Thickness (m) :"; color "Color [RGB] :"; opacity "Opacity (0...1) :"
      mask help: This block creates a flat, single, square tile element. The square tile body is mass-less, so it will not have an effect on the dynamic simulation. This square tile element can be used as a graphic reference by itself, or as part of a composite graphic reference made of an array of interconnected tiles. The square tile is aligned with the XY plane, and the block provides frame connector ports to the middle points on each of the four sides of the body of the square - right (+X), left (-X), top (+Y) and bottom (-Y). All dimensions are in meters.
      settings: PortSchema="{\"entries\":[{\"content\":{\"sides\":[{\"content\":{\"connectorIds\":[\"LConn1\"]},\"type\":\"ConnectorPlacement.EquallySpacedRectSide\",\"uuid\":\"a971723f-ea37-4e9b-910b-501b94fb0ba2\"},{\"content\":{\"connectorIds\":[\"RConn1\"],\"side\":\"RIGHT\"},\"type\":\"ConnectorPlacement.EquallySpacedRectSide\",\"uuid\":\"e50175c1-005c-4b0b-bced-b882197eaab2\"},{\"content\":{\"connectorIds\":[\"LConn2\"],\"side\":\"TOP\"},\"type\":\"ConnectorPlacement.EquallySpacedRectSide\",\"uuid\":\"2a04a964-d53e-47ee-8c79-d53dd599bafe\"},{\"content\":{\"connectorIds\":[\"RConn2\"],\"side\":\"BOTTOM\"},\"type\":\"ConnectorPlacement.EquallySpacedRectSide\",\"uuid\":\"a0066dd6-a193-491c-afbe-bac00dfc3505\"}]},\"type\":\"ConnectorPlacement.EquallySpacedConnector\",\"uuid\":\"c80211c6-bb24-481b-97ca-2752015f3b18\"}],\"packageUris\":[\"http://schema.mathworks.com/mf0/Connector/19700101\"],\"version\":\"1.0\"}"
  Tile166 : Subsystem  mask(Square Tile){side=side, thickness=thick, color=color1, opacity=opacity}
      mask prompts: side "Side (m) :"; thickness "Thickness (m) :"; color "Color [RGB] :"; opacity "Opacity (0...1) :"
      mask help: This block creates a flat, single, square tile element. The square tile body is mass-less, so it will not have an effect on the dynamic simulation. This square tile element can be used as a graphic reference by itself, or as part of a composite graphic reference made of an array of interconnected tiles. The square tile is aligned with the XY plane, and the block provides frame connector ports to the middle points on each of the four sides of the body of the square - right (+X), left (-X), top (+Y) and bottom (-Y). All dimensions are in meters.
      settings: PortSchema="{\"entries\":[{\"content\":{\"sides\":[{\"content\":{\"connectorIds\":[\"LConn1\"]},\"type\":\"ConnectorPlacement.EquallySpacedRectSide\",\"uuid\":\"a971723f-ea37-4e9b-910b-501b94fb0ba2\"},{\"content\":{\"connectorIds\":[\"RConn1\"],\"side\":\"RIGHT\"},\"type\":\"ConnectorPlacement.EquallySpacedRectSide\",\"uuid\":\"e50175c1-005c-4b0b-bced-b882197eaab2\"},{\"content\":{\"connectorIds\":[\"LConn2\"],\"side\":\"TOP\"},\"type\":\"ConnectorPlacement.EquallySpacedRectSide\",\"uuid\":\"2a04a964-d53e-47ee-8c79-d53dd599bafe\"},{\"content\":{\"connectorIds\":[\"RConn2\"],\"side\":\"BOTTOM\"},\"type\":\"ConnectorPlacement.EquallySpacedRectSide\",\"uuid\":\"a0066dd6-a193-491c-afbe-bac00dfc3505\"}]},\"type\":\"ConnectorPlacement.EquallySpacedConnector\",\"uuid\":\"c80211c6-bb24-481b-97ca-2752015f3b18\"}],\"packageUris\":[\"http://schema.mathworks.com/mf0/Connector/19700101\"],\"version\":\"1.0\"}"
  Tile167 : Subsystem  mask(Square Tile){side=side, thickness=thick, color=color2, opacity=opacity}
      mask prompts: side "Side (m) :"; thickness "Thickness (m) :"; color "Color [RGB] :"; opacity "Opacity (0...1) :"
      mask help: This block creates a flat, single, square tile element. The square tile body is mass-less, so it will not have an effect on the dynamic simulation. This square tile element can be used as a graphic reference by itself, or as part of a composite graphic reference made of an array of interconnected tiles. The square tile is aligned with the XY plane, and the block provides frame connector ports to the middle points on each of the four sides of the body of the square - right (+X), left (-X), top (+Y) and bottom (-Y). All dimensions are in meters.
      settings: PortSchema="{\"entries\":[{\"content\":{\"sides\":[{\"content\":{\"connectorIds\":[\"LConn1\"]},\"type\":\"ConnectorPlacement.EquallySpacedRectSide\",\"uuid\":\"a971723f-ea37-4e9b-910b-501b94fb0ba2\"},{\"content\":{\"connectorIds\":[\"RConn1\"],\"side\":\"RIGHT\"},\"type\":\"ConnectorPlacement.EquallySpacedRectSide\",\"uuid\":\"e50175c1-005c-4b0b-bced-b882197eaab2\"},{\"content\":{\"connectorIds\":[\"LConn2\"],\"side\":\"TOP\"},\"type\":\"ConnectorPlacement.EquallySpacedRectSide\",\"uuid\":\"2a04a964-d53e-47ee-8c79-d53dd599bafe\"},{\"content\":{\"connectorIds\":[\"RConn2\"],\"side\":\"BOTTOM\"},\"type\":\"ConnectorPlacement.EquallySpacedRectSide\",\"uuid\":\"a0066dd6-a193-491c-afbe-bac00dfc3505\"}]},\"type\":\"ConnectorPlacement.EquallySpacedConnector\",\"uuid\":\"c80211c6-bb24-481b-97ca-2752015f3b18\"}],\"packageUris\":[\"http://schema.mathworks.com/mf0/Connector/19700101\"],\"version\":\"1.0\"}"
  Tile168 : Subsystem  mask(Square Tile){side=side, thickness=thick, color=color1, opacity=opacity}
      mask prompts: side "Side (m) :"; thickness "Thickness (m) :"; color "Color [RGB] :"; opacity "Opacity (0...1) :"
      mask help: This block creates a flat, single, square tile element. The square tile body is mass-less, so it will not have an effect on the dynamic simulation. This square tile element can be used as a graphic reference by itself, or as part of a composite graphic reference made of an array of interconnected tiles. The square tile is aligned with the XY plane, and the block provides frame connector ports to the middle points on each of the four sides of the body of the square - right (+X), left (-X), top (+Y) and bottom (-Y). All dimensions are in meters.
      settings: PortSchema="{\"entries\":[{\"content\":{\"sides\":[{\"content\":{\"connectorIds\":[\"LConn1\"]},\"type\":\"ConnectorPlacement.EquallySpacedRectSide\",\"uuid\":\"a971723f-ea37-4e9b-910b-501b94fb0ba2\"},{\"content\":{\"connectorIds\":[\"RConn1\"],\"side\":\"RIGHT\"},\"type\":\"ConnectorPlacement.EquallySpacedRectSide\",\"uuid\":\"e50175c1-005c-4b0b-bced-b882197eaab2\"},{\"content\":{\"connectorIds\":[\"LConn2\"],\"side\":\"TOP\"},\"type\":\"ConnectorPlacement.EquallySpacedRectSide\",\"uuid\":\"2a04a964-d53e-47ee-8c79-d53dd599bafe\"},{\"content\":{\"connectorIds\":[\"RConn2\"],\"side\":\"BOTTOM\"},\"type\":\"ConnectorPlacement.EquallySpacedRectSide\",\"uuid\":\"a0066dd6-a193-491c-afbe-bac00dfc3505\"}]},\"type\":\"ConnectorPlacement.EquallySpacedConnector\",\"uuid\":\"c80211c6-bb24-481b-97ca-2752015f3b18\"}],\"packageUris\":[\"http://schema.mathworks.com/mf0/Connector/19700101\"],\"version\":\"1.0\"}"
  Tile169 : Subsystem  mask(Square Tile){side=side, thickness=thick, color=color2, opacity=opacity}
      mask prompts: side "Side (m) :"; thickness "Thickness (m) :"; color "Color [RGB] :"; opacity "Opacity (0...1) :"
      mask help: This block creates a flat, single, square tile element. The square tile body is mass-less, so it will not have an effect on the dynamic simulation. This square tile element can be used as a graphic reference by itself, or as part of a composite graphic reference made of an array of interconnected tiles. The square tile is aligned with the XY plane, and the block provides frame connector ports to the middle points on each of the four sides of the body of the square - right (+X), left (-X), top (+Y) and bottom (-Y). All dimensions are in meters.
      settings: PortSchema="{\"entries\":[{\"content\":{\"sides\":[{\"content\":{\"connectorIds\":[\"LConn1\"]},\"type\":\"ConnectorPlacement.EquallySpacedRectSide\",\"uuid\":\"a971723f-ea37-4e9b-910b-501b94fb0ba2\"},{\"content\":{\"connectorIds\":[\"RConn1\"],\"side\":\"RIGHT\"},\"type\":\"ConnectorPlacement.EquallySpacedRectSide\",\"uuid\":\"e50175c1-005c-4b0b-bced-b882197eaab2\"},{\"content\":{\"connectorIds\":[\"LConn2\"],\"side\":\"TOP\"},\"type\":\"ConnectorPlacement.EquallySpacedRectSide\",\"uuid\":\"2a04a964-d53e-47ee-8c79-d53dd599bafe\"},{\"content\":{\"connectorIds\":[\"RConn2\"],\"side\":\"BOTTOM\"},\"type\":\"ConnectorPlacement.EquallySpacedRectSide\",\"uuid\":\"a0066dd6-a193-491c-afbe-bac00dfc3505\"}]},\"type\":\"ConnectorPlacement.EquallySpacedConnector\",\"uuid\":\"c80211c6-bb24-481b-97ca-2752015f3b18\"}],\"packageUris\":[\"http://schema.mathworks.com/mf0/Connector/19700101\"],\"version\":\"1.0\"}"
  Tile17 : Subsystem  mask(Square Tile){side=side, thickness=thick, color=color1, opacity=opacity}
      mask prompts: side "Side (m) :"; thickness "Thickness (m) :"; color "Color [RGB] :"; opacity "Opacity (0...1) :"
      mask help: This block creates a flat, single, square tile element. The square tile body is mass-less, so it will not have an effect on the dynamic simulation. This square tile element can be used as a graphic reference by itself, or as part of a composite graphic reference made of an array of interconnected tiles. The square tile is aligned with the XY plane, and the block provides frame connector ports to the middle points on each of the four sides of the body of the square - right (+X), left (-X), top (+Y) and bottom (-Y). All dimensions are in meters.
      settings: PortSchema="{\"entries\":[{\"content\":{\"sides\":[{\"content\":{\"connectorIds\":[\"LConn1\"]},\"type\":\"ConnectorPlacement.EquallySpacedRectSide\",\"uuid\":\"a971723f-ea37-4e9b-910b-501b94fb0ba2\"},{\"content\":{\"connectorIds\":[\"RConn1\"],\"side\":\"RIGHT\"},\"type\":\"ConnectorPlacement.EquallySpacedRectSide\",\"uuid\":\"e50175c1-005c-4b0b-bced-b882197eaab2\"},{\"content\":{\"connectorIds\":[\"LConn2\"],\"side\":\"TOP\"},\"type\":\"ConnectorPlacement.EquallySpacedRectSide\",\"uuid\":\"2a04a964-d53e-47ee-8c79-d53dd599bafe\"},{\"content\":{\"connectorIds\":[\"RConn2\"],\"side\":\"BOTTOM\"},\"type\":\"ConnectorPlacement.EquallySpacedRectSide\",\"uuid\":\"a0066dd6-a193-491c-afbe-bac00dfc3505\"}]},\"type\":\"ConnectorPlacement.EquallySpacedConnector\",\"uuid\":\"c80211c6-bb24-481b-97ca-2752015f3b18\"}],\"packageUris\":[\"http://schema.mathworks.com/mf0/Connector/19700101\"],\"version\":\"1.0\"}"
  Tile170 : Subsystem  mask(Square Tile){side=side, thickness=thick, color=color2, opacity=opacity}
